simulink library "xbsIndex_r3"  (Simulink 6.1)
PreLoadFcn:
  | xlmeta;
undefined symbols (not defined in the file or in its folder): sim_pause
libraries: xbsIndex_r3 x62, simulink x1
(part 1 of 4)
settings Model: Creator=arvinds  LastModifiedBy=milne

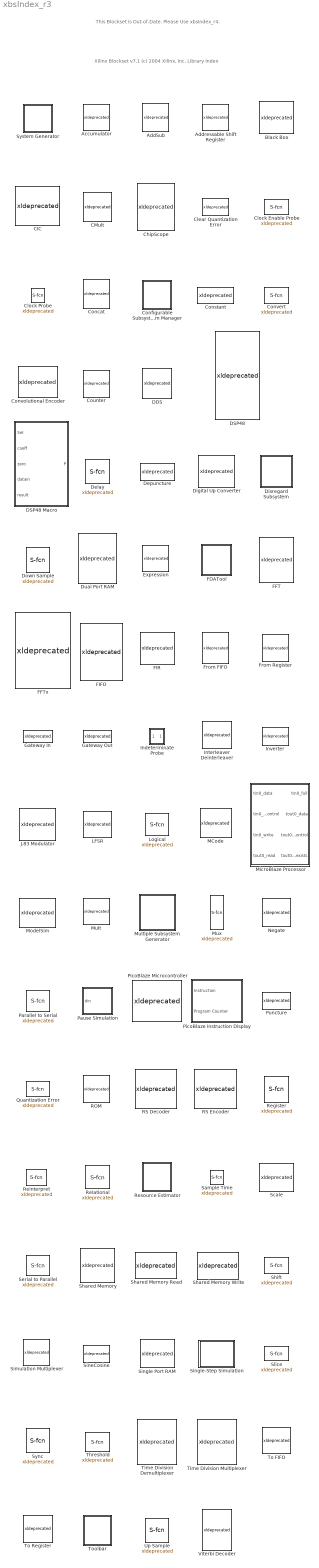
== system xbsIndex_r3 ==
  note: Xilinx Blockset v7.1
      | (c) 2004 Xilinx, Inc.
      |
      | Library Index
  note: This Blockset is Out-of-Date.
      | Please Use xbsIndex_r4.
  " System Generator" : Subsystem  Tag=genX  mask(Xilinx System Generator){xilinxfamily=Virtex2, part=xc2v1000, speed=-4, package=bg575, synthesis_tool=XST, directory=./netlist, testbench=off, simulink_period=1, sysclk_period=100, incr_netlist=off, trim_vbits=Everywhere in SubSystem, dbl_ovrd=According to Block Masks, core_generation=According to Block Masks, run_coregen=off, deprecated_control=off, eval_field=0}
      mask prompts: xilinxfamily "Xilinx Family"; synthesis_tool "Synthesis Tool"; directory "Target Directory"; simulink_period "Simulink Period"; sysclk_period "System Clock Period"; incr_netlist "Incremental Netlisting"; trim_vbits "Trim Valid Bits"; dbl_ovrd "Override with Doubles"; core_generation "Generate Cores"; run_coregen "Run CoreGen"; deprecated_control "Show Deprecated Controls"; eval_field "Evaluation Field"
      mask help: Interface to the Xilinx System Generator to generate HDL code for the subsystem hierarchy in which the block resides. The block also gives coarse grain (subsystem wide) control over capabilities such as overriding with doubles. Double click on the icon to access these features.
      mask init:
      | [bg,fg]=xlcmap_r3('SGen');
      | iPos = get_param(gcb,'Position');
      | iWidth=iPos(3)-iPos(1); iHeight=iPos(4)-iPos(2);
      | iCx=iWidth/2;
      | iCy=iHeight/2;
      | [logoX, logoY] = xlogo(iPos);
      settings: AttributesFormatString=System\nGenerator  OpenFcn=modelName = get_param(bdroot, 'name');h = errordlg(sprintf(['This block is from an outdated copy of the Xilinx Blockset.\nPlease run xlUpdateModel(''' modelName ''') to update this design.']), 'Update Required');
      mask Help: eval('xlWeb(xlhtmldoclink('' System Generator''))');
      mask StyleString: edit,edit,edit,edit,popup(Spectrum|Synplify|Synplify Pro|XST),edit,checkbox,edit,edit,checkbox,popup(According to Block Masks|Everywhere in SubSystem|No Where in SubSystem),popup(According to Block Masks|Everywhere in SubSystem|No Where in SubSystem),popup(According to Block Masks|Everywhere Available|Not Needed - Already Generated),checkbox,checkbox,edit
      mask Display:
      | patch([0 iWidth iWidth 0],[0 0 iHeight iHeight] , bg);
      | patch(logoX,logoY, fg);
      | ;plot([0 0 iWidth iWidth 0], [0 iHeight iHeight 0 0]);
  Accumulator : S-Function  FunctionName=xldeprecated  Parameters=nin,nout  mask(Xilinx Accumulator){n_bits=8, overflow=Wrap, operation=Add, scale=1, explicit_period=off, period=1, rst=on, hasbypass=off, en=off, dbl_ovrd=off, show_param=off, gen_core=off, use_rpm=on, xl_area=[0, 0, 0, 0, 0, 0, 0], xl_use_area=off}
      mask prompts: n_bits "Number of Output Bits"; scale "Feedback Scaling"; explicit_period "Use Explicit Sample Period"; period "Sample Period  (use -1 to inherit first known input period)"; rst "Provide Reset Port"; hasbypass "Reinitialize with Input 'b' on Reset"; en "Provide Enable Port"; dbl_ovrd "Override with Doubles"; show_param "---------------------- Show Implementation Parameters -----------------------------------------------------------------------------------"; gen_core "Generate Core"; use_rpm "Use Placement Information for Core"; xl_area "FPGA Area [Slices, FFs, BRAMs, LUTs, IOBs, Emb. Mults, TBUFs]"; xl_use_area "Use Area Above For Estimation"
      mask help:
      | BLOCK IS OUT OF DATE.
      |
      | This block is from an outdated copy of the Xilinx Blockset. Please run xlUpdateModel('<model-name>') to update to the latest version.
      mask init:
      | [designRoot, family, part, speed, package, simulinkPeriod, sysclkPeriod, dbl_ovrd, trimVbit] = xlSysgenSettings(gcb,1,1);
      | [bg,fg] = xlcmap_r3('XBlock',dbl_ovrd);
      | iPos = get_param(gcb,'Position');
      | iWidth=iPos(3)-iPos(1); iHeight=iPos(4)-iPos(2);
      | iCx=iWidth/2;
      | iCy=iHeight/2;
      | [logoX, logoY] = xlogo(iPos);
      | [enPortNum,enPortStr,rstPortNum,rstPortStr] = xlport_en_rst(en,rst,2);
      | 
      | % one time added for param list
      | hasRST = rst;
      | hasEN =  en;
      | dblOvrd = dbl_ovrd;
      | nbits = n_bits;
      | precision0 = 1;
      | useCore = 1;
      | gen_core = 1;
      | latency = 1;
      | explicitClk = explicit_period;
      | 
      | % just pass everything to s-function
      | sfcn_mwsv__ = get_param(gcb, 'MaskWSVariables');
      | 
      | nport = get_param(gcbh, 'ports');
      | nin = nport(1);
      | nout = nport(2);
      mask Help: eval('xlWeb(xlhtmldoclink(''Accumulator''))');
      mask StyleString: edit,popup(Wrap|Saturate|Error),popup(Add|Subtract),popup(1|1/2|1/4|1/8|1/16|1/32|1/64|1/128|1/256),checkbox,edit,checkbox,checkbox,checkbox,checkbox,checkbox,checkbox,checkbox,edit,checkbox
      mask Display:
      | patch([0 iWidth iWidth 0],[0 0 iHeight iHeight] , bg);
      | patch(logoX,logoY , fg);
      | port_label('output',1,'q');
      | port_label('input',1,'b');
      | port_label('input',enPortNum,enPortStr);
      | port_label('input',rstPortNum,rstPortStr);
      | ;plot([0 0 iWidth iWidth 0], [0 iHeight iHeight 0 0]);
  AddSub : S-Function  FunctionName=xldeprecated  Parameters=nin,nout  mask(Xilinx Adder/Subtractor){mode=Addition, precision=Full, arith_type=Unsigned, n_bits=8, bin_pt=2, quantization=Truncate, overflow=Wrap, latency=0, explicit_period=off, period=1, use_carryin=off, use_carryout=off, en=off, dbl_ovrd=off, show_param=off, use_core=on, pipeline=off, use_rpm=on, gen_core=off, xl_area=[0, 0, 0, 0, 0, 0, 0], xl_use_area=off}
      mask prompts: arith_type "Output Type"; n_bits "Number of Bits"; bin_pt "Binary Point"; explicit_period "Use Explicit Sample Period"; period "Sample Period  (use -1 to inherit first known input period)"; use_carryin "Provide Carry-in Port"; use_carryout "Provide Carry-out Port"; en "Provide Enable Port"; dbl_ovrd "Override with Doubles"; show_param "---------------------- Show Implementation Parameters -----------------------------------------------------------------------------------"; use_core "Implement with Xilinx Smart-IP Core"; pipeline "Pipeline to Greatest Extent Possible"; use_rpm "Use Placement Information for Core"; gen_core "Generate Core"; xl_area "FPGA Area [Slices, FFs, BRAMs, LUTs, IOBs, Emb. Mults, TBUFs]"; xl_use_area "Use Area Above For Estimation"
      mask help:
      | BLOCK IS OUT OF DATE.
      |
      | This block is from an outdated copy of the Xilinx Blockset. Please run xlUpdateModel('<model-name>') to update to the latest version.
      mask init:
      | rst = 0;
      | cin_port = 1; cin_str = 'a';
      | cout_port = 1; cout_str = '';
      | nextport = 3;
      | if(use_carryin)
      | 	cin_port = 3;
      | 	cin_str = 'cin';
      | 	nextport = 4;
      | end
      | if(use_carryout)
      | 	cout_port = 2;
      | 	cout_str = 'cout';
      | end
      | if (mode ~= 3)
      |    [enPortNum,enPortStr,rstPortNum,rstPortStr] = xlport_en_rst(en,rst,nextport);
      | else
      |   [enPortNum,enPortStr,rstPortNum,rstPortStr] = xlport_en_rst(en,rst,nextport+1);
      | end
      | 
      | [designRoot, family, part, speed, package, simulinkPeriod, sysclkPeriod, dbl_ovrd, trimVbit] = xlSysgenSettings(gcb,1,1);
      | mprt=1; mstr=''; ostr2='';
      | if (mode==1)
      |   ostr = 'a+b';
      | elseif (mode==2)
      |   ostr = 'a-b';
      | else
      |   ostr = 'a+b';
      |   ostr2 = '_b';
      |   if(use_carryin)
      |      mprt=4; 
      |   else
      | 	 mprt = 3;
      |   end
      |   mstr='sub';
      | end
      | zstr=''; zpstr='';
      | if latency > 0
      |   zstr = 'z';
      |   zpstr = sprintf('-%d', latency);
      | end
      | [bg,fg] = xlcmap_r3('XBlock',dbl_ovrd);
      | iPos = get_param(gcb,'Position');
      | iWidth=iPos(3)-iPos(1); iHeight=iPos(4)-iPos(2);
      | iCx=iWidth/2;
      | iCy=iHeight/2;
      | [logoX, logoY] = xlogo(iPos);
      | zstrx = 0.45*iWidth-3; if (zstrx<3) zstrx=3; end
      | zstry = 0.36*iHeight-7; if (zstry<3) zstry=3; end
      | 
      | 
      | % one time added for param list
      | dblOvrd = dbl_ovrd;
      | useCore = use_core;
      | precision0 = precision;
      | precision1 = precision;
      | z0 = [n_bits bin_pt arith_type quantization overflow];
      | z1 = [1 0 1 1 1];
      | explicitClk = explicit_period;
      | gen_core = 1;
      | hasRST = rst;
      | hasEN = en;
      | 
      | % just pass everything to s-function
      | sfcn_mwsv__ = get_param(gcb, 'MaskWSVariables');
      | 
      | nport = get_param(gcbh, 'ports');
      | nin = nport(1);
      | nout = nport(2);
      mask Help: eval('xlWeb(xlhtmldoclink(''AddSub''))');
      mask StyleString: popup(Addition|Subtraction|Addition or Subtraction),popup(Full|User Defined),popup(Unsigned|Signed  (2's comp)),edit,edit,popup(Truncate|Round  (unbiased: +/- Inf)),popup(Wrap|Saturate|Error),edit,checkbox,edit,checkbox,checkbox,checkbox,checkbox,checkbox,checkbox,checkbox,checkbox,checkbox,edit,checkbox
      mask Display:
      | patch([0 iWidth iWidth 0],[0 0 iHeight iHeight] , bg);
      | patch(logoX,logoY , fg);
      | text(zstrx,zstry,zstr);
      | text(zstrx+5,zstry+5,zpstr);
      | port_label('output',1,ostr);
      | port_label('output',1,ostr2);
      | port_label('output',cout_port,cout_str);
      | port_label('input',mprt,mstr)
      | port_label('input',1,'a');
      | port_label('input',2,'b');
      | port_label('input',cin_port,cin_str);
      | port_label('input',enPortNum,enPortStr);
      | ;plot([0 0 iWidth iWidth 0], [0 iHeight iHeight 0 0]);
  Addressable Shift Register : S-Function  FunctionName=xldeprecated  Parameters=nin,nout  mask(Xilinx Addressable Shift Register){infer_latency=on, depth=2, initVector=[0], explicit_period=off, period=1, accept_only_valid=off, en=off, dbl_ovrd=off, show_param=off, use_rpm=on, gen_core=off, xl_area=[0, 0, 0, 0, 0, 0, 0], xl_use_area=off}
      mask prompts: infer_latency "Infer Maximum Latency (depth) Using Address Port Width"; depth "Maximum Latency (depth)"; initVector "Initial Value Vector"; explicit_period "Use Explicit Sample Period"; period "Sample Period  (use -1 to inherit first known input period)"; accept_only_valid "Shift In Only Valid Data"; en "Provide Enable Port"; dbl_ovrd "Override with Doubles"; show_param "---------------------- Show Implementation Parameters -----------------------------------------------------------------------------------"; use_rpm "Use Placement Information for Core"; gen_core "Generate Core"; xl_area "FPGA Area [Slices, FFs, BRAMs, LUTs, IOBs, Emb. Mults, TBUFs]"; xl_use_area "Use Area Above For Estimation"
      mask help:
      | BLOCK IS OUT OF DATE.
      |
      | This block is from an outdated copy of the Xilinx Blockset. Please run xlUpdateModel('<model-name>') to update to the latest version.
      mask init:
      | % get enable port number and string
      | [enPortNum, enPortStr] =xlport_en_rst(en,0,3);
      | 
      | [designRoot, family, part, speed, package, simulinkPeriod, sysclkPeriod, dbl_ovrd, trimVbit] = xlSysgenSettings(gcb,1,1);
      | [bg,fg] = xlcmap_r3('XBlock',dbl_ovrd);
      | iPos = get_param(gcb,'Position');
      | iWidth=iPos(3)-iPos(1); iHeight=iPos(4)-iPos(2);
      | iCx=iWidth/2;
      | iCy=iHeight/2;
      | [logoX, logoY] = xlogo(iPos);
      | 
      | 
      | 
      | 
      | % one time added for param list
      | init = initVector;
      | useCore = 1;
      | dblOvrd = dbl_ovrd;
      | vOnly = accept_only_valid;
      | precision0 = 1;
      | explicitClk = explicit_period;
      | hasEN = en;
      | gen_core = 1;
      | rpm = use_rpm;
      | 
      | % just pass everything to s-function
      | sfcn_mwsv__ = get_param(gcb, 'MaskWSVariables');
      | 
      | nport = get_param(gcbh, 'ports');
      | nin = nport(1);
      | nout = nport(2);
      mask Help: eval('xlWeb(xlhtmldoclink(''Addressable Shift Register''))');
      mask Display:
      | patch([0 iWidth iWidth 0],[0 0 iHeight iHeight] , bg);
      | patch(logoX,logoY , fg);
      | port_label('input', 1,'d');
      | port_label('input', 2,'addr');
      | port_label('input',enPortNum,enPortStr);
      | port_label('output',1,'q');
      | 
      | ;plot([0 0 iWidth iWidth 0], [0 iHeight iHeight 0 0]);
  Black Box : S-Function  FunctionName=xldeprecated  Parameters=nin,nout  mask(Xilinx Blackbox Block){init_code=, sim_method=Inactive, engine_block=, show_param=off, xl_area=[0, 0, 0, 0, 0, 0, 0], xl_use_area=off}
      mask prompts: init_code "Block Configuration M-Function"; sim_method "Simulation Mode"; engine_block "HDL Co-Simulator To Use  (specify helper block by name)"; show_param "---------------------- Show Implementation Parameters -----------------------------------------------------------------------------------"; xl_area "FPGA Area [Slices, FFs, BRAMs, LUTs, IOBs, Emb. Mults, TBUFs]"; xl_use_area "Use Area Above For Estimation"
      mask help:
      | BLOCK IS OUT OF DATE.
      |
      | This block is from an outdated copy of the Xilinx Blockset. Please run xlUpdateModel('<model-name>') to update to the latest version.
      mask init:
      | [designRoot, family, part, speed, package, simulinkPeriod, sysclkPeriod, dbl_ovrd, trimVbit] = xlSysgenSettings(gcb,0,0);
      | 
      | [bg,fg] = xlcmap_r3('XBlock');
      | iPos = get_param(gcb,'Position');
      | iWidth=iPos(3)-iPos(1); iHeight=iPos(4)-iPos(2);
      | iCx=iWidth/2;
      | iCy=iHeight/2;
      | [logoX, logoY] = xlogo(iPos);
      | zstr='z'; zpstr='-1';
      | zstrx = iCx-3; if (zstrx<16) zstr='';zpstr=''; end
      | zstry = iCy;
      | 
      | precision0 = 1;
      | latency = 0;
      | dblOvrd = 0;
      | 
      | mdlPath = xlGetMdlDir(bdroot);
      | 
      | refBlk = get_param(gcb,'referenceBlock');
      | if (isempty(refBlk) | strncmp(refBlk,'xbsIndex',8))
      | 	srcPath = mdlPath;
      | else
      | 	srcPath = xlPathToReference;
      | 	if (isempty(srcPath))
      | 		srcPath = mdlPath;
      | 	end
      | end
      | 
      | if (sim_method==2)
      | 	validEngineBlock = 0;
      | 	try
      | 	  engineBlock = xlBlockNameRelPath(get_param(gcb,'Parent'),engine_block);
      | 	catch
      | 	  engineBlock = '//';
      | 	end
      | 	try 
      | 	  engineWorkDir = get_param(engineBlock,'dir');
      | 	  validEngineBlock = 1;
      | 	catch
      | 	end
      | end
      | 
      | % just pass everything to s-function
      | sfcn_mwsv__ = get_param(gcb, 'MaskWSVariables');
      | 
      | plabel = xlbbPortLabelStruct(gcb,init_code,mdlPath);
      | 
      | nport = get_param(gcbh, 'ports');
      | nin = nport(1);
      | nout = nport(2);
      mask Help: eval('xlWeb(xlhtmldoclink(''Black Box''))');
      mask StyleString: edit,popup(Inactive|Use HDL Co-Simulation),edit,checkbox,edit,checkbox
      mask Display:
      | patch([0 iWidth iWidth 0],[0 0 iHeight iHeight] , bg);
      | patch(logoX,logoY, fg);
      | plot([0 0 iWidth iWidth 0], [0 iHeight iHeight 0 0]);
      |   port_label(plabel.d1,plabel.i1,plabel.n1);
      |   port_label(plabel.d2,plabel.i2,plabel.n2);
      |   port_label(plabel.d3,plabel.i3,plabel.n3);
      |   port_label(plabel.d4,plabel.i4,plabel.n4);
      |   port_label(plabel.d5,plabel.i5,plabel.n5);
      |   port_label(plabel.d6,plabel.i6,plabel.n6);
      |   port_label(plabel.d7,plabel.i7,plabel.n7);
      |   port_label(plabel.d8,plabel.i8,plabel.n8);
      |   port_label(plabel.d9,plabel.i9,plabel.n9);
      |   port_label(plabel.d10,plabel.i10,plabel.n10);
      |   port_label(plabel.d11,plabel.i11,plabel.n11);
      |   port_label(plabel.d12,plabel.i12,plabel.n12);
      |   port_label(plabel.d13,plabel.i13,plabel.n13);
      |   port_label(plabel.d14,plabel.i14,plabel.n14);
      |   port_label(plabel.d15,plabel.i15,plabel.n15);
      |   port_label(plabel.d16,plabel.i16,plabel.n16);
      |   port_label(plabel.d17,plabel.i17,plabel.n17);
      |   port_label(plabel.d18,plabel.i18,plabel.n18);
      |   port_label(plabel.d19,plabel.i19,plabel.n19);
      |   port_label(plabel.d20,plabel.i20,plabel.n20);
      |   port_label(plabel.d21,plabel.i21,plabel.n21);
      |   port_label(plabel.d22,plabel.i22,plabel.n22);
      |   port_label(plabel.d23,plabel.i23,plabel.n23);
      |   port_label(plabel.d24,plabel.i24,plabel.n24);
      |   port_label(plabel.d25,plabel.i25,plabel.n25);
      |   port_label(plabel.d26,plabel.i26,plabel.n26);
      |   port_label(plabel.d27,plabel.i27,plabel.n27);
      |   port_label(plabel.d28,plabel.i28,plabel.n28);
      |   port_label(plabel.d29,plabel.i29,plabel.n29);
      |   port_label(plabel.d30,plabel.i30,plabel.n30);
      |   port_label(plabel.d31,plabel.i31,plabel.n31);
      |   port_label(plabel.d32,plabel.i32,plabel.n32);
      |   port_label(plabel.d33,plabel.i33,plabel.n33);
      |   port_label(plabel.d34,plabel.i34,plabel.n34);
      |   port_label(plabel.d35,plabel.i35,plabel.n35);
      |   port_label(plabel.d36,plabel.i36,plabel.n36);
      |   port_label(plabel.d37,plabel.i37,plabel.n37);
      |   port_label(plabel.d38,plabel.i38,plabel.n38);
      |   port_label(plabel.d39,plabel.i39,plabel.n39);
      |   port_label(plabel.d40,plabel.i40,plabel.n40);
      |   port_label(plabel.d41,plabel.i41,plabel.n41);
      |   port_label(plabel.d42,plabel.i42,plabel.n42);
      |   port_label(plabel.d43,plabel.i43,plabel.n43);
      |   port_label(plabel.d44,plabel.i44,plabel.n44);
      |   port_label(plabel.d45,plabel.i45,plabel.n45);
      |   port_label(plabel.d46,plabel.i46,plabel.n46);
      |   port_label(plabel.d45,plabel.i45,plabel.n45);
      |   port_label(plabel.d48,plabel.i48,plabel.n48);
      |   port_label(plabel.d49,plabel.i49,plabel.n49);
      |   port_label(plabel.d50,plabel.i50,plabel.n50);
      |   port_label(plabel.d51,plabel.i51,plabel.n51);
      |   port_label(plabel.d52,plabel.i52,plabel.n52);
      |   port_label(plabel.d53,plabel.i53,plabel.n53);
      |   port_label(plabel.d54,plabel.i54,plabel.n54);
      |   port_label(plabel.d55,plabel.i55,plabel.n55);
      |   port_label(plabel.d56,plabel.i56,plabel.n56);
      |   port_label(plabel.d57,plabel.i57,plabel.n57);
      |   port_label(plabel.d58,plabel.i58,plabel.n58);
      |   port_label(plabel.d59,plabel.i59,plabel.n59);
      |   port_label(plabel.d60,plabel.i60,plabel.n60);
      |   port_label(plabel.d61,plabel.i61,plabel.n61);
      |   port_label(plabel.d62,plabel.i62,plabel.n62);
      |   port_label(plabel.d63,plabel.i63,plabel.n63);
      |   port_label(plabel.d64,plabel.i64,plabel.n64);
  CIC : S-Function  FunctionName=xldeprecated  Parameters=nin,nout  mask(Xilinx Cascaded Integrator-Comb Filter){filter_type=Decimator, samp_rate_change=8, stages=2, differential_delay=1, latency=1, explicit_period=off, period=1, dbl_ovrd=off, show_param=off, use_rpm=on, gen_core=off, xl_area=[0, 0, 0, 0, 0, 0, 0], xl_use_area=off}
      mask prompts: filter_type "Filter Type"; samp_rate_change "Sample Rate Change"; stages "Number of Stages"; differential_delay "Differential Delay"; explicit_period "Use Explicit Sample Period"; period "Sample Period"; dbl_ovrd "Override with Doubles"; show_param "---------------------- Show Implementation Parameters -----------------------------------------------------------------------------------"; use_rpm "Use Placement Information for Core"; gen_core "Generate Core"; xl_area "FPGA Area [Slices, FFs, BRAMs, LUTs, IOBs, Emb. Mults, TBUFs]"; xl_use_area "Use Area Above For Estimation"
      mask help:
      | BLOCK IS OUT OF DATE.
      |
      | This block is from an outdated copy of the Xilinx Blockset. Please run xlUpdateModel('<model-name>') to update to the latest version.
      mask init:
      | [designRoot, family, part, speed, package, simulinkPeriod, sysclkPeriod, dbl_ovrd, trimVbit] = xlSysgenSettings(gcb,1,0);
      | trimVbit=1;
      | [bg,fg] = xlcmap_r3('XBlock',dbl_ovrd);
      | iPos = get_param(gcb,'Position');
      | iWidth=iPos(3)-iPos(1); iHeight=iPos(4)-iPos(2);
      | iCx=iWidth/2;
      | iCy=iHeight/2;
      | [logoX, logoY] = xlogo(iPos);
      | if(filter_type == 1)
      | str = sprintf('%d-Stage CIC\n1:%d Interpolator',stages,samp_rate_change);
      |      aw = 3;
      |      ah = 7;
      |      arrowX = [0, (-aw), (-aw), 0, 0, (1), (1), (aw+1), (aw+1), (1)];
      |      arrowY = [(ah-1), (ah-aw-1), (ah-aw), (ah), (-ah), (-ah), (ah), (ah-aw), (ah-aw-1),(ah-1)];
      |      arrowX = arrowX + iCx - 1 - 3.5*length(str);
      |      arrowY = arrowY + iCy + 3;
      | else
      | str = sprintf('%d-Stage CIC\n%d:1 Decimator',stages,samp_rate_change);
      |      aw = 3;
      |      ah = 7;
      |      arrowX = [0, (-aw), (-aw), 0, 0, (1), (1), (aw+1), (aw+1), (1)];
      |     arrowY = [(ah-1), (ah-aw-1), (ah-aw), (ah), (-ah), (-ah), (ah), (ah-aw), (ah-aw-1), (ah-1)];
      |     arrowX = arrowX + iCx - 2 - 3.5*length(str);
      |     arrowY = iCy - arrowY + 2;
      | end
      | 
      | % one time added for param list
      | rate_change = samp_rate_change;
      | diff_delay = differential_delay;
      | create_rpm = use_rpm;
      | dblOvrd = dbl_ovrd;
      | useCore = 1;
      | precision0 = 1;
      | precision1 = 1;
      | explicitClk = explicit_period;
      | gen_core = 1;
      | 
      | % just pass everything to s-function
      | sfcn_mwsv__ = get_param(gcb, 'MaskWSVariables');
      | 
      | nport = get_param(gcbh, 'ports');
      | nin = nport(1);
      | nout = nport(2);
      mask Help: eval('xlWeb(xlhtmldoclink(''CIC''))');
      mask StyleString: popup(Interpolator|Decimator),edit,edit,popup(1|2),edit,checkbox,edit,checkbox,checkbox,checkbox,checkbox,edit,checkbox
      mask Display:
      | patch([0 iWidth iWidth 0],[0 0 iHeight iHeight] , bg);
      | patch(logoX,logoY , fg);
      | disp(str);
      | plot([0 0 iWidth iWidth 0], [0 iHeight iHeight 0 0]);
      | 
      | port_label('input',1,'xn');
      | port_label('input',2,'vin');
      | 
      | port_label('output',1,'yn');
      | port_label('output',2,'vout');
  CMult : S-Function  FunctionName=xldeprecated  Parameters=nin,nout  mask(Xilinx Constant Multiplier){const=1, show_cparam=off, const_n_bits=8, const_bin_pt=6, show_output_param=off, precision=Full, arith_type=Signed  (2's comp), n_bits=8, bin_pt=6, quantization=Round  (unbiased: +/- Inf), overflow=Wrap, latency=0, explicit_period=off, period=1, en=off, dbl_ovrd=off, show_param=off, mult_type=Parallel, oversample=2, mem_type=Distributed RAM, pipeline=off, use_rpm=on, placement_style=Rectangular Shape, gen_core=off, xl_area=[0, 0, 0, 0, 0, 0, 0], xl_use_area=off}
      mask prompts: const "Value of Constant"; show_cparam "---------------------- Show Constant Data Type Parameters ---------------------------------------------------------"; const_n_bits "Number of Bits in Constant"; const_bin_pt "Binary Point of Constant"; show_output_param "---------------------- Show Output Data Type Parameters ------------------------------"; arith_type "Output Type"; n_bits "Number of Bits"; bin_pt "Binary Point"; explicit_period "Use Explicit Sample Period"; period "Sample Period  (use -1 to inherit first known input period)"; en "Provide Enable Port"; dbl_ovrd "Override with Doubles"; show_param "---------------------- Show Implementation Parameters -----------------------------------------------------------------------------------"; mult_type "Multiplier Type"; oversample "Hardware Over-Sampling Rate"; mem_type "Memory Type"; pipeline "Pipeline to Greatest Extent Possible"; use_rpm "Use Placement Information for Core"; placement_style "Placement Style"; gen_core "Generate Core"; xl_area "FPGA Area [Slices, FFs, BRAMs, LUTs, IOBs, Emb. Mults, TBUFs]"; xl_use_area "Use Area Above For Estimation"
      mask help:
      | BLOCK IS OUT OF DATE.
      |
      | This block is from an outdated copy of the Xilinx Blockset. Please run xlUpdateModel('<model-name>') to update to the latest version.
      mask init:
      | rst = 0;
      | [enPortNum,enPortStr,rstPortNum,rstPortStr] = xlport_en_rst(en,rst,2);
      | 
      | multtype = mult_type;
      | if (multtype == 2)
      |   osamp = oversample;
      | else
      |   osamp = 1;
      | end
      | mprt = 1; ostr='';
      | mprt_loadb = 1; ostr_loadb='';
      | const_arith_type = (const<0) + 1;
      | [designRoot, family, part, speed, package, simulinkPeriod, sysclkPeriod, dbl_ovrd, trimVbit] = xlSysgenSettings(gcb,1,1);
      | k = xltodouble(const, const_n_bits, const_bin_pt, const_arith_type, 2, 2);
      | if (k<0)
      |   str = sprintf('x (%0.4g)',k);
      | else
      |   str = sprintf('x %0.4g',k);
      | end
      | zstr=''; zpstr='';
      | if latency > 0
      |   zstr = 'z';
      |   zpstr = sprintf('-%d', latency);
      | end
      | [bg,fg] = xlcmap_r3('XBlock',dbl_ovrd);
      | iPos = get_param(gcb,'Position');
      | iWidth=iPos(3)-iPos(1); iHeight=iPos(4)-iPos(2);
      | iCx=iWidth/2;
      | iCy=iHeight/2;
      | [logoX, logoY] = xlogo(iPos);
      | logoX = logoX*.54 + 2;
      | logoY = logoY*.54+ iHeight*.23;
      | zstrx = 15;
      | zstry = 0.36*iHeight-4; if (zstry<3) zstry=3; end
      | 
      | 
      | 
      | % one time added for param list
      | dblOvrd = dbl_ovrd;
      | useCore = 1;
      | precision0 = precision;
      | z0 = [n_bits bin_pt arith_type quantization overflow];
      | coef = const;
      | ctype = [const_n_bits const_bin_pt const_arith_type 2 2];
      | explicitClk = explicit_period;
      | memtype = mem_type;
      | reload = 0;
      | oversample = osamp;
      | gen_core = 1;
      | rpm = use_rpm;
      | style = placement_style;
      | hasRST = rst;
      | hasEN = en;
      | 
      | % just pass everything to s-function
      | sfcn_mwsv__ = get_param(gcb, 'MaskWSVariables');
      | 
      | nport = get_param(gcbh, 'ports');
      | nin = nport(1);
      | nout = nport(2);
      mask Help: eval('xlWeb(xlhtmldoclink(''CMult''))');
      mask StyleString: edit,checkbox,edit,edit,checkbox,popup(Full|User Defined),popup(Unsigned|Signed  (2's comp)),edit,edit,popup(Truncate|Round  (unbiased: +/- Inf)),popup(Wrap|Saturate|Flag as Error),edit,checkbox,edit,checkbox,checkbox,checkbox,popup(Parallel|Sequential),edit,popup(Distributed RAM|Block RAM),checkbox,checkbox,popup(Rectangular Shape|Triangular Packing),checkbox,edit,checkbox
      mask Display:
      | patch([0 iWidth 0],[0 iCy iHeight] , bg);
      | patch(logoX,logoY , fg);
      | plot([0 iWidth 0 0],[0 iCy iHeight 0] );
      | text(zstrx,zstry,zstr);
      | text(zstrx+4,zstry+4,zpstr);
      | port_label('output',1,[str  '  ']);
      | port_label('input',enPortNum,enPortStr);
  ChipScope : S-Function  Tag=chipScopeGenerate  FunctionName=xldeprecated  Parameters=nin,nout  mask(Xilinx ChipScope Core){num_trig_ports=2, show_trig_port=0, match_units_t0=1, match_type_t0=Basic, match_units_t1=1, match_type_t1=Basic, match_units_t2=1, match_type_t2=Basic, match_units_t3=1, match_type_t3=Basic, match_units_t4=1, match_type_t4=Basic, match_units_t5=1, match_type_t5=Basic, match_units_t6=1, match_type_t6=Basic, match_units_t7=1, match_type_t7=Basic, match_units_t8=1, match_type_t8=Basic, match_units_t9=3, match_type_t9=Basic, match_units_t10=1, match_type_t10=Basic, match_units_t11=1, match_type_t11=Basic, match_units_t12=1, match_type_t12=Basic, match_units_t13=1, match_type_t13=Basic, match_units_t14=1, match_type_t14=Basic, match_units_t15=1, match_type_t15=Basic, data_is_trigger=off, num_data_ports=1, data_depth=512, SRL16s=on, explicit_period=off, period=-1, dbl_ovrd=off}
      mask prompts: num_trig_ports "Number of Trigger Ports"; show_trig_port "Display Options for Trigger Port"; match_units_t0 "Number of Match Units for Trigger Port 0"; match_type_t0 "Match Type of Trigger Port 0"; match_units_t1 "Number of Match Units for Trigger Port 1"; match_type_t1 "Match Type of Trigger Port 1"; match_units_t2 "Number of Match Units for Trigger Port 2"; match_type_t2 "Match Type of Trigger Port 2"; match_units_t3 "Number of Match Units for Trigger Port 3"; match_type_t3 "Match Type of Trigger Port 3"; match_units_t4 "Number of Match Units for Trigger Port 4"; match_type_t4 "Match Type of Trigger Port 4"; match_units_t5 "Number of Match Units for Trigger Port 5"; match_type_t5 "Match Type of Trigger Port 5"; match_units_t6 "Number of Match Units for Trigger Port 6"; match_type_t6 "Match Type of Trigger Port 6"; match_units_t7 "Number of Match Units for Trigger Port 7"; match_type_t7 "Match Type of Trigger Port 7"; match_units_t8 "Number of Match Units for Trigger Port 8"; match_type_t8 "Match Type of Trigger Port 8"; match_units_t9 "Number of Match Units for Trigger Port 9"; match_type_t9 "Match Type of Trigger Port 9"; match_units_t10 "Number of Match Units for Trigger Port 10"; match_type_t10 "Match Type of Trigger Port 10"; match_units_t11 "Number of Match Units for Trigger Port 11"; match_type_t11 "Match Type of Trigger Port 11"; match_units_t12 "Number of Match Units for Trigger Port 12"; match_type_t12 "Match Type of Trigger Port 12"; match_units_t13 "Number of Match Units for Trigger Port 13"; match_type_t13 "Match Type of Trigger Port 13"; match_units_t14 "Number of Match Units for Trigger Port 14"; match_type_t14 "Match Type of Trigger Port 14"; match_units_t15 "Number of Match Units for Trigger Port 15"; match_type_t15 "Match Type of Trigger Port 15"; data_is_trigger "Use Trigger Ports as Data"; num_data_ports "Number of Data Ports"; data_depth "Depth of Capture Buffer"; SRL16s "Use SRL16s ( when possible)"; explicit_period "Use Explicit Sample Period"; period "Sample Period  (use -1 to inherit first known input period)"; dbl_ovrd "Override with Doubles"
      mask help:
      | BLOCK IS OUT OF DATE.
      |
      | This block is from an outdated copy of the Xilinx Blockset. Please run xlUpdateModel('<model-name>') to update to the latest version.
      mask init:
      | try
      | 
      | [designRoot, family, part, speed, package, simulinkPeriod, sysclkPeriod, dbl_ovrd, trimVbit] = xlSysgenSettings(gcb,1,1);
      | if isempty(family)
      | 	family = 'Virtex2';
      | end;
      | [xldirectory, xlSynthTool] = xlFindTargetDir(gcb);
      | xlISEVer = xlGetISEVer;
      | sysgen_root = fileparts(fileparts(which('sysgen')));
      | 
      | [bg,fg] = xlcmap_r3('XBlock',dbl_ovrd);
      | iPos = get_param(gcb,'Position');
      | iWidth=iPos(3)-iPos(1); iHeight=iPos(4)-iPos(2);
      | iCx=iWidth/2;
      | iCy=iHeight/2;
      | [logoX, logoY] = xlogo(iPos);
      | 
      | if (data_is_trigger == 1)
      | 	numDataPorts = 0;
      | else
      | 	numDataPorts = num_data_ports;
      | end;
      | inputs = num_trig_ports + numDataPorts;
      | dprt = [1:inputs ones(1,144-inputs)];
      | for i = 1:144
      | 	dstr{i} = ''; 
      | end;
      | 
      | % Set trigger port names
      | for i = 1:num_trig_ports
      | 	if (data_is_trigger == 1)
      | 		dstr{i} = ['trig' num2str(i-1) '/data' num2str(i-1)];
      | 	else
      | 		dstr{i} = ['trig' num2str(i-1)]; 
      | 	end;
      | end;
      | 
      | % Set data port names
      | for i = 1:numDataPorts
      | 	dstr{i+num_trig_ports} = ['data' num2str(i-1)];
      | end;
      | 
      | % Replace default names with signal names
      | signalNames = xlInputSignalNames(gcb);
      | for i = 1:length(signalNames)
      | 	if ~isempty(signalNames{i})
      | 		dstr{i} = signalNames{i};
      | 	end;
      | end;
      | 
      | % one time added for param list
      | latency = 1;
      | precision0 = 1;
      | dblOvrd = 0;
      | 
      | % just pass everything to s-function
      | sfcn_mwsv__ = get_param(gcb, 'MaskWSVariables');
      | 
      | catch
      | 	disp(lasterr);
      | end;
      | nport = get_param(gcbh, 'ports');
      | nin = nport(1);
      | nout = nport(2);
      mask Help: eval('xlWeb(xlhtmldoclink(''ChipScope''))');
      mask StyleString: popup(1|2|3|4|5|6|7|8|9|10|11|12|13|14|15|16),popup(0|1|2|3|4|5|6|7|8|9|10|11|12|13|14|15),popup(1|2|3|4),popup(Basic|Basic With Edges|Extended|Extended With Edges|Range|Range With Edges),popup(1|2|3|4),popup(Basic|Basic With Edges|Extended|Extended With Edges|Range|Range With Edges),popup(1|2|3|4),popup(Basic|Basic With Edges|Extended|Extended With edges|Range|Range With Edges),popup(1|2|3|4),popup(Basic|Basic With Edges|Extended|Extended With Edges|Range|Range With Edges),popup(1|2|3|4),popup(Basic|Basic With Edges|Extended|Extended With Edges|Range|Range With Edges),popup(1|2|3|4),popup(Basic|Basic With Edges|Extended|Extended With Edges|Range|Range with Edges),popup(1|2|3|4),popup(Basic|Basic With Edges|Extended|Extended With Edges|Range|Range With Edges),popup(1|2|3|4),popup(Basic|Basic With Edges|Extended|Extended With Edges|Range|Range With Edges),popup(1|2|3|4),popup(Basic|Basic With Edges|Extended|Extended With Edges|Range|Range With Edges),popup(1|2|3|4),popup(Basic|Basic With Edges|Extended|Extended With Edges|Range|Range With Edges),popup(1|2|3|4),popup(Basic|Basic With Edges|Extended|Extended with Edges|Range|Range With Edges),popup(1|2|3|4),popup(Basic|Basic With Edges|Extended|Extended With Edges|Range|Range With Edges),popup(1|2|3|4),popup(Basic|Basic With Edges|Extended|Extended With Edges|Range|Range With Edges),popup(1|2|3|4),popup(Basic|Basic With Edges|Extended|Extended With Edges|Range|Range With Edges),popup(1|2|3|4),popup(Basic|Basic With Edges|Extended|Extended With Edges|Range|Range With Edges),popup(1|2|3|4),popup(Basic|Basic With edges|Extended|Extended With Edges|Range|Range With Edges),checkbox,edit,popup(512|1024|2048|4096|8192|16384),checkbox,checkbox,edit,checkbox
      mask Display:
      | patch([0 iWidth iWidth 0],[0 0 iHeight iHeight] , bg);
      | patch(logoX,logoY, fg);
      | ;plot([0 0 iWidth iWidth 0], [0 iHeight iHeight 0 0]);
      | 
      | port_label('input',dprt(1),dstr{1});
      | port_label('input',dprt(2),dstr{2});
      | port_label('input',dprt(3),dstr{3});
      | port_label('input',dprt(4),dstr{4});
      | port_label('input',dprt(5),dstr{5});
      | port_label('input',dprt(6),dstr{6});
      | port_label('input',dprt(7),dstr{7});
      | port_label('input',dprt(8),dstr{8});
      | port_label('input',dprt(9),dstr{9});
      | port_label('input',dprt(10),dstr{10});
      | port_label('input',dprt(11),dstr{11});
      | port_label('input',dprt(12),dstr{12});
      | port_label('input',dprt(13),dstr{13});
      | port_label('input',dprt(14),dstr{14});
      | port_label('input',dprt(15),dstr{15});
      | port_label('input',dprt(16),dstr{16});
      | port_label('input',dprt(17),dstr{17});
      | port_label('input',dprt(18),dstr{18});
      | port_label('input',dprt(19),dstr{19});
      | port_label('input',dprt(20),dstr{20});
      | port_label('input',dprt(21),dstr{21});
      | port_label('input',dprt(22),dstr{22});
      | port_label('input',dprt(23),dstr{23});
      | port_label('input',dprt(24),dstr{24});
      | port_label('input',dprt(25),dstr{25});
      | port_label('input',dprt(26),dstr{26});
      | port_label('input',dprt(27),dstr{27});
      | port_label('input',dprt(28),dstr{28});
      | port_label('input',dprt(29),dstr{29});
      | port_label('input',dprt(30),dstr{30});
      | port_label('input',dprt(31),dstr{31});
      | port_label('input',dprt(32),dstr{32});
      | port_label('input',dprt(33),dstr{33});
      | port_label('input',dprt(34),dstr{34});
      | port_label('input',dprt(35),dstr{35});
      | port_label('input',dprt(36),dstr{36});
      | port_label('input',dprt(37),dstr{37});
      | port_label('input',dprt(38),dstr{38});
      | port_label('input',dprt(39),dstr{39});
      | port_label('input',dprt(40),dstr{40});
      | port_label('input',dprt(41),dstr{41});
      | port_label('input',dprt(42),dstr{42});
      | port_label('input',dprt(43),dstr{43});
      | port_label('input',dprt(44),dstr{44});
      | port_label('input',dprt(45),dstr{45});
      | port_label('input',dprt(46),dstr{46});
      | port_label('input',dprt(47),dstr{47});
      | port_label('input',dprt(48),dstr{48});
      | port_label('input',dprt(49),dstr{49});
      | port_label('input',dprt(50),dstr{50});
      | port_label('input',dprt(51),dstr{51});
      | port_label('input',dprt(52),dstr{52});
      | port_label('input',dprt(53),dstr{53});
      | port_label('input',dprt(54),dstr{54});
      | port_label('input',dprt(55),dstr{55});
      | port_label('input',dprt(56),dstr{56});
      | port_label('input',dprt(57),dstr{57});
      | port_label('input',dprt(58),dstr{58});
      | port_label('input',dprt(59),dstr{59});
      | port_label('input',dprt(60),dstr{60});
      | port_label('input',dprt(61),dstr{61});
      | port_label('input',dprt(62),dstr{62});
      | port_label('input',dprt(63),dstr{63});
      | port_label('input',dprt(64),dstr{64});
      | port_label('input',dprt(65),dstr{65});
      | port_label('input',dprt(66),dstr{66});
      | port_label('input',dprt(67),dstr{67});
      | port_label('input',dprt(68),dstr{68});
      | port_label('input',dprt(69),dstr{69});
      | port_label('input',dprt(70),dstr{70});
      | port_label('input',dprt(71),dstr{71});
      | port_label('input',dprt(72),dstr{72});
      | port_label('input',dprt(73),dstr{73});
      | port_label('input',dprt(74),dstr{74});
      | port_label('input',dprt(75),dstr{75});
      | port_label('input',dprt(76),dstr{76});
      | port_label('input',dprt(77),dstr{77});
      | port_label('input',dprt(78),dstr{78});
      | port_label('input',dprt(79),dstr{79});
      | port_label('input',dprt(80),dstr{80});
      | port_label('input',dprt(81),dstr{81});
      | port_label('input',dprt(82),dstr{82});
      | port_label('input',dprt(83),dstr{83});
      | port_label('input',dprt(84),dstr{84});
      | port_label('input',dprt(85),dstr{85});
      | port_label('input',dprt(86),dstr{86});
      | port_label('input',dprt(87),dstr{87});
      | port_label('input',dprt(88),dstr{88});
      | port_label('input',dprt(89),dstr{89});
      | port_label('input',dprt(90),dstr{90});
      | port_label('input',dprt(91),dstr{91});
      | port_label('input',dprt(92),dstr{92});
      | port_label('input',dprt(93),dstr{93});
      | port_label('input',dprt(94),dstr{94});
      | port_label('input',dprt(95),dstr{95});
      | port_label('input',dprt(96),dstr{96});
      | port_label('input',dprt(97),dstr{97});
      | port_label('input',dprt(98),dstr{98});
      | port_label('input',dprt(99),dstr{99});
      | port_label('input',dprt(100),dstr{100});
      | port_label('input',dprt(101),dstr{101});
      | port_label('input',dprt(102),dstr{102});
      | port_label('input',dprt(103),dstr{103});
      | port_label('input',dprt(104),dstr{104});
      | port_label('input',dprt(105),dstr{105});
      | port_label('input',dprt(106),dstr{106});
      | port_label('input',dprt(107),dstr{107});
      | port_label('input',dprt(108),dstr{108});
      | port_label('input',dprt(109),dstr{109});
      | port_label('input',dprt(110),dstr{110});
      | port_label('input',dprt(111),dstr{111});
      | port_label('input',dprt(112),dstr{112});
      | port_label('input',dprt(113),dstr{113});
      | port_label('input',dprt(114),dstr{114});
      | port_label('input',dprt(115),dstr{115});
      | port_label('input',dprt(116),dstr{116});
      | port_label('input',dprt(117),dstr{117});
      | port_label('input',dprt(118),dstr{118});
      | port_label('input',dprt(119),dstr{119});
      | port_label('input',dprt(120),dstr{120});
      | port_label('input',dprt(121),dstr{121});
      | port_label('input',dprt(122),dstr{122});
      | port_label('input',dprt(123),dstr{123});
      | port_label('input',dprt(124),dstr{124});
      | port_label('input',dprt(125),dstr{125});
      | port_label('input',dprt(126),dstr{126});
      | port_label('input',dprt(127),dstr{127});
      | port_label('input',dprt(128),dstr{128});
      | port_label('input',dprt(129),dstr{129});
      | port_label('input',dprt(130),dstr{130});
      | port_label('input',dprt(131),dstr{131});
      | port_label('input',dprt(132),dstr{132});
      | port_label('input',dprt(133),dstr{133});
      | port_label('input',dprt(134),dstr{134});
      | port_label('input',dprt(135),dstr{135});
      | port_label('input',dprt(136),dstr{136});
      | port_label('input',dprt(137),dstr{137});
      | port_label('input',dprt(138),dstr{138});
      | port_label('input',dprt(139),dstr{139});
      | port_label('input',dprt(140),dstr{140});
      | port_label('input',dprt(141),dstr{141});
      | port_label('input',dprt(142),dstr{142});
      | port_label('input',dprt(143),dstr{143});
      | port_label('input',dprt(144),dstr{144});
  Clear Quantization Error : S-Function  FunctionName=xldeprecated  Parameters=nin,nout  mask(Xilinx Clear Quantization Error Block){opt_port=off}
      mask prompts: opt_port "Add Optional Clear Port"
      mask help:
      | BLOCK IS OUT OF DATE.
      |
      | This block is from an outdated copy of the Xilinx Blockset. Please run xlUpdateModel('<model-name>') to update to the latest version.
      mask init:
      | [designRoot, family, part, speed, package, simulinkPeriod, sysclkPeriod, dbl_ovrd, trimVbit] = xlSysgenSettings(gcb,0,2);
      | [bg,fg] = xlcmap_r3('XBlock',dbl_ovrd);
      | iPos = get_param(gcb,'Position');
      | iWidth=iPos(3)-iPos(1); iHeight=iPos(4)-iPos(2);
      | iCx=iWidth/2;
      | iCy=iHeight/2;
      | [logoX, logoY] = xlogo(iPos);
      | if (opt_port==0)
      |   pnum=1;
      |   pstr='';
      | else
      |   pnum=2;
      |   pstr='*clrE';
      | end
      | 
      | % one time added for param list
      | precision0 = 1;
      | has_clr_pin = opt_port;
      | dblOvrd = dbl_ovrd;
      | 
      | % just pass everything to s-function
      | sfcn_mwsv__ = get_param(gcb, 'MaskWSVariables');
      | 
      | nport = get_param(gcbh, 'ports');
      | nin = nport(1);
      | nout = nport(2);
      mask Help: eval('xlWeb(xlhtmldoclink(''Clear Quantization Error''))');
      mask Display:
      | patch([0 iWidth iWidth 0],[0 0 iHeight iHeight] , bg);
      | patch(logoX,logoY , fg);
      | port_label('input',pnum,pstr);
      | port_label('output',1,'clr err');
      | ;plot([0 0 iWidth iWidth 0], [0 iHeight iHeight 0 0]);
  Clock Enable Probe : S-Function  FunctionName=xldeprecated  Parameters=nin,nout  mask(Xilinx Clock Enable Probe){}
      mask help:
      | BLOCK IS OUT OF DATE.
      |
      | This block is from an outdated copy of the Xilinx Blockset. Please run xlUpdateModel('<model-name>') to update to the latest version.
      mask init:
      | [designRoot, family, part, speed, package, simulinkPeriod, sysclkPeriod] = xlSysgenSettings(gcb,0,0);
      | 
      | [bg,fg] = xlcmap_r3('XBlock',0);
      | iPos = get_param(gcb,'Position');
      | iWidth=iPos(3)-iPos(1); iHeight=iPos(4)-iPos(2);
      | iCx=iWidth/2;
      | iCy=iHeight/2;
      | [logoX, logoY] = xlogo(iPos);
      | 
      | % one time added for param list
      | precision0 = 1;
      | dblOvrd = 0;
      | trimVbit = 0;
      | 
      | % just pass everything to s-function
      | sfcn_mwsv__ = get_param(gcb, 'MaskWSVariables');
      | 
      | nport = get_param(gcbh, 'ports');
      | nin = nport(1);
      | nout = nport(2);
      mask Help: eval('xlWeb(xlhtmldoclink(''Clock Enable Probe''))');
      mask Display:
      | patch([0 iWidth iWidth 0],[0 0 iHeight iHeight] , bg);
      | patch(logoX,logoY, fg);
      | ;plot([0 0 iWidth iWidth 0], [0 iHeight iHeight 0 0]);
      | 
      | disp('CE');
  Clock Probe : S-Function  FunctionName=xldeprecated  Parameters=nin,nout  mask(Xilinx Clock Probe){}
      mask help:
      | BLOCK IS OUT OF DATE.
      |
      | This block is from an outdated copy of the Xilinx Blockset. Please run xlUpdateModel('<model-name>') to update to the latest version.
      mask init:
      | [designRoot, family, part, speed, package, simulinkPeriod, sysclkPeriod, dbl_ovrd, trimVbit] = xlSysgenSettings(gcb,0,0);
      | 
      | [bg,fg] = xlcmap_r3('IO');
      | iPos = get_param(gcb,'Position');
      | iWidth=iPos(3)-iPos(1); iHeight=iPos(4)-iPos(2);
      | iCx=iWidth/2;
      | iCy=iHeight/2;
      | shapeX = iCx* (1 + cos(0:pi/6:2*pi));
      | shapeY = iCy* (1 + sin(0:pi/6:2*pi));
      | 
      | % just pass everything to s-function
      | sfcn_mwsv__ = get_param(gcb, 'MaskWSVariables');
      | 
      | nport = get_param(gcbh, 'ports');
      | nin = nport(1);
      | nout = nport(2);
      mask Help: eval('xlWeb(xlhtmldoclink(''Clock Probe''))');
      mask Display:
      | patch(shapeX,shapeY, bg);
      | plot(shapeX,shapeY);
      | disp('CLK');
  Concat : S-Function  FunctionName=xldeprecated  Parameters=nin,nout  mask(Xilinx Bus Concatenator){num_inputs=2, explicit_period=off, period=1, dbl_ovrd=off}
      mask prompts: num_inputs "Number of Inputs"; explicit_period "Use Explicit Sample Period"; period "Sample Period  (use -1 to inherit first known input period)"; dbl_ovrd "Override with Doubles"
      mask help:
      | BLOCK IS OUT OF DATE.
      |
      | This block is from an outdated copy of the Xilinx Blockset. Please run xlUpdateModel('<model-name>') to update to the latest version.
      mask init:
      | [designRoot, family, part, speed, package, simulinkPeriod, sysclkPeriod, dbl_ovrd, trimVbit] = xlSysgenSettings(gcb,1,1);
      | [bg,fg] = xlcmap_r3('XBlock',dbl_ovrd);
      | iPos = get_param(gcb,'Position');
      | iWidth=iPos(3)-iPos(1); iHeight=iPos(4)-iPos(2);
      | iCx=iWidth/2;
      | iCy=iHeight/2;
      | [logoX, logoY] = xlogo(iPos);
      | 
      | 
      | 
      | 
      | % one time added for param list
      | numInputs = num_inputs + 1;
      | precision0 = 1;
      | latency = 0;
      | dblOvrd = dbl_ovrd;
      | explicitClk = explicit_period;
      | 
      | 
      | % just pass everything to s-function
      | sfcn_mwsv__ = get_param(gcb, 'MaskWSVariables');
      | 
      | nport = get_param(gcbh, 'ports');
      | nin = nport(1);
      | nout = nport(2);
      mask Help: eval('xlWeb(xlhtmldoclink(''Concat''))');
      mask StyleString: popup(2|3|4|5|6|7|8|9|10|11|12|13|14|15|16),checkbox,edit,checkbox
      mask Display:
      | patch([0 iWidth iWidth 0],[0 0 iHeight iHeight] , bg);
      | patch(logoX,logoY, fg);
      | port_label('input',1,'hi');
      | port_label('input',num_inputs+1,'lo');
      | port_label('output',1,'cat');
      | ;plot([0 0 iWidth iWidth 0], [0 iHeight iHeight 0 0]);
  Configurable Subsystem Manager : Subsystem  Tag=xcfgMgr  mask(Xilinx System Generator){}
      mask help: Interface to the Xilinx System Generator to generate HDL code for the subsystem hierarchy in which the block resides. The block also gives coarse grain (subsystem wide) control over capabilities such as overriding with doubles. Double click on the icon to access these features.
      mask init:
      | [bg, fg] = xlcmap_r3('XTool');
      | 
      | %[bg1, fg] = xlcmap_r3('XBlock',0);
      | iPos = get_param(gcb,'Position');
      | iWidth=iPos(3)-iPos(1); iHeight=iPos(4)-iPos(2);
      | iCx=iWidth/2;
      | iCy=iHeight/2;
      | [logoX, logoY] = xlogo(iPos);
      settings: AttributesFormatString=Configurable Subsystem\nManager  OpenFcn=modelName = get_param(bdroot, 'name');h = errordlg(sprintf(['This block is from an outdated copy of the Xilinx Blockset.\nPlease run xlUpdateModel(''' modelName ''') to update this design.']), 'Update Required');
      mask Help: eval('xlWeb(xlhtmldoclink(''Configurable Subsystem Manager''))');
      mask Display:
      | patch([0 iWidth iWidth 0],[0 0 iHeight iHeight] , bg);
      | patch(logoX,logoY , fg);
      | ;plot([0 0 iWidth iWidth 0], [0 iHeight iHeight 0 0]);
  Constant : S-Function  FunctionName=xldeprecated  Parameters=nin,nout  mask(Xilinx Constant Block){const=1, equ=P=C, arith_type=Unsigned, n_bits=1, bin_pt=0, opselect=C, inp2=PCIN>>17, opr=+, inp1=P, carry=CIN, iostate=0, explicit_period=off, period=1, dbl_ovrd=off}
      mask prompts: const "Constant Value"; equ "DSP48 operation"; arith_type "Type"; n_bits "Number of Bits"; bin_pt "Binary Point Position"; opselect "Operation Select"; inp2 "Z Mux"; opr "Operand"; inp1 "YX Muxes"; carry "Carry Input"; explicit_period "Sampled Constant"; period "Sample Period"; dbl_ovrd "Override with Double"
      mask help:
      | BLOCK IS OUT OF DATE.
      |
      | This block is from an outdated copy of the Xilinx Blockset. Please run xlUpdateModel('<model-name>') to update to the latest version.
      mask init:
      | [designRoot, family, part, speed, package, simulinkPeriod, sysclkPeriod, dbl_ovrd, trimVbit] = xlSysgenSettings(gcb,1,2);
      | [bg,fg]=xlcmap_r3('XBlock',dbl_ovrd);
      | iPos = get_param(gcb,'Position');
      | iWidth=iPos(3)-iPos(1); iHeight=iPos(4)-iPos(2);
      | nchar = floor(iWidth/7.0);
      | op = 0;
      | dsp48instr = 0;
      | if (arith_type==1)
      |   bool = 1;
      |   k= xltodouble(const,1,0,1,2,2);
      |   format_str = sprintf('%%0.%dg',nchar);
      |   str = sprintf(format_str,k);
      |   if (length(str)+3<nchar)
      |   	str = ['k =' str];
      |   end
      | elseif (arith_type == 4) %dsp48
      |   dsp48instr = 1;
      |   bool = 0;
      |   str = equ;
      |   n_bits = 11;
      |   bin_pt = 0;
      |   arith_type = 1;
      |   [op,opmode, sub, carryin, carryin_sel] = xlcalcDSP48Op(equ);
      | else
      |   bool = 0;
      |   arith_type=arith_type-1;
      |   k= xltodouble(const,n_bits,bin_pt,arith_type,2,2);
      |   format_str = sprintf('%%0.%dg',nchar);
      |   str = sprintf(format_str,k);
      |   if (length(str)+3<nchar)
      |     str = ['k =' str];
      |   end
      | end
      | 
      | 
      | iCx=iWidth/2;
      | iCy=iHeight/2;
      | [logoX, logoY] = xlogo(iPos);
      | 
      | 
      | % one time added for param list
      | dblOvrd = dbl_ovrd;
      | precision0 = 2;
      | z0 = [n_bits bin_pt arith_type 2 2];
      | explicitClk = explicit_period;
      | 
      | 
      | % just pass everything to s-function
      | sfcn_mwsv__ = get_param(gcb, 'MaskWSVariables');
      | 
      | nport = get_param(gcbh, 'ports');
      | nin = nport(1);
      | nout = nport(2);
      mask Help: eval('xlWeb(xlhtmldoclink(''Constant''))');
      mask StyleString: edit,edit,popup(Boolean|Unsigned|Signed  (2's comp)|DSP48 Instruction),edit,edit,popup(C + A*B|PCIN + A*B|P + A*B|A * B|C + A:B|C - A:B|C|custom),popup(0|PCIN|P|C|PCIN>>17|P>>17),popup(+|-),popup(0|P|A:B|A*B|C|P+C|A:B+C),popup(0|1|CIN|~SIGN(P or PCIN)|~SIGN(A*B or A:B)|~SIGND(A*B or A:B)),edit,checkbox,edit,checkbox
      mask Display:
      | patch([0 iWidth iWidth 0],[0 0 iHeight iHeight] , bg);
      | patch(logoX,logoY , fg);
      | port_label('output',1,str);
      | ;plot([0 0 iWidth iWidth 0], [0 iHeight iHeight 0 0]);
  Convert : S-Function  FunctionName=xldeprecated  Parameters=nin,nout  mask(Xilinx Converter Block){arith_type=Signed  (2's comp), n_bits=8, bin_pt=6, quantization=Truncate, overflow=Wrap, latency=0, explicit_period=off, period=1, dbl_ovrd=off, show_param=off, inserted_by_tool=off, pipeline=off, xl_area=[0, 0, 0, 0, 0, 0, 0], xl_use_area=off}
      mask prompts: arith_type "Output Type"; n_bits "Number of Bits"; bin_pt "Binary Point"; quantization "Quantization Behavior"; overflow "Overflow Behavior"; explicit_period "Use Explicit Sample Period"; period "Sample Period"; dbl_ovrd "Override with Doubles"; show_param "---------------------- Show Implementation Parameters -----------------------------------------------------------------------------------"; inserted_by_tool "Hidden Parameter:  inserted_by_tool"; pipeline "Pipeline to Greatest Extent Possible"; xl_area "FPGA Area [Slices, FFs, BRAMs, LUTs, IOBs, Emb. Mults, TBUFs]"; xl_use_area "Use Area Above For Estimation"
      mask help:
      | BLOCK IS OUT OF DATE.
      |
      | This block is from an outdated copy of the Xilinx Blockset. Please run xlUpdateModel('<model-name>') to update to the latest version.
      mask init:
      | [designRoot, family, part, speed, package, simulinkPeriod, sysclkPeriod, dbl_ovrd, trimVbit] = xlSysgenSettings(gcb,1,1);
      | if (arith_type==1)
      |   bool = 1;
      | else
      |   bool = 0;
      |   arith_type = arith_type-1;
      | end
      | zstr=''; zpstr='';
      | if latency > 0
      |   zstr = 'z';
      |   zpstr = sprintf('-%d', latency);
      | end
      | [bg,fg] = xlcmap_r3('XBlock',dbl_ovrd);
      | if (inserted_by_tool)
      |   bg = [1.00 0.50 0.25];
      | end
      | iPos = get_param(gcb,'Position');
      | iWidth=iPos(3)-iPos(1); iHeight=iPos(4)-iPos(2);
      | iCx=iWidth/2;
      | iCy=iHeight/2;
      | [logoX, logoY] = xlogo(iPos);
      | zstrx = 0.45*iWidth-11; if (zstrx<3) zstrx=3; end
      | zstry = 0.36*iHeight-7; if (zstry<3) zstry=3; end
      | 
      | 
      | % one time added for param list
      | dblOvrd = dbl_ovrd;
      | precision0 = 2;
      | z0 = [n_bits bin_pt arith_type quantization overflow];
      | explicitClk = explicit_period;
      | 
      | 
      | % just pass everything to s-function
      | sfcn_mwsv__ = get_param(gcb, 'MaskWSVariables');
      | 
      | nport = get_param(gcbh, 'ports');
      | nin = nport(1);
      | nout = nport(2);
      mask Help: eval('xlWeb(xlhtmldoclink(''Convert''))');
      mask StyleString: popup(Boolean|Unsigned|Signed  (2's comp)),edit,edit,popup(Truncate|Round  (unbiased: +/- Inf)|Round  (unbiased: Even Values)),popup(Wrap|Saturate|Error),edit,checkbox,edit,checkbox,checkbox,checkbox,checkbox,edit,checkbox
      mask Display:
      | patch([0 iWidth iWidth 0],[0 0 iHeight iHeight] , bg);
      | patch(logoX,logoY , fg);
      | text(zstrx,zstry,zstr);
      | text(zstrx+5,zstry+5,zpstr);
      | port_label('output',1,'cast');
      | plot([0 0 iWidth iWidth 0], [0 iHeight iHeight 0 0]);
  Convolutional Encoder : S-Function  FunctionName=xldeprecated  Parameters=nin,nout  mask(Xilinx Convolutional Encoder){clength=3, conv_codes=[7 5 6], explicit_period=off, period=1, rst=off, en=off, dbl_ovrd=off, show_param=off, use_rpm=on, gen_core=off, xl_area=[0, 0, 0, 0, 0, 0, 0], xl_use_area=off}
      mask prompts: clength "Constraint Length"; conv_codes "Convolution Code Array (octal)"; explicit_period "Use Explicit Sample Period"; period "Sample Period  (use -1 to inherit first known input period)"; rst "Provide Reset Port"; en "Provide Enable Port"; dbl_ovrd "Override with Doubles"; show_param "---------------------- Show Implementation Parameters -----------------------------------------------------------------------------------"; use_rpm "Use Placement Information for Core"; gen_core "Generate Core"; xl_area "FPGA Area [Slices, FFs, BRAMs, LUTs, IOBs, Emb. Mults, TBUFs]"; xl_use_area "Use Area Above For Estimation"
      mask help:
      | BLOCK IS OUT OF DATE.
      |
      | This block is from an outdated copy of the Xilinx Blockset. Please run xlUpdateModel('<model-name>') to update to the latest version.
      mask init:
      | numstr3 = 2;
      | numstr4 = 2;
      | numstr5 = 2;
      | numstr6 = 2;
      | numstr7 = 2;
      | outstr3 = ''; outstr4 = ''; outstr5 = ''; outstr6 = ''; outstr7 = '';
      | [enPortNum,enPortStr,rstPortNum,rstPortStr] = xlport_en_rst(en,rst,3);
      | code_struct = xlconvertcodes(clength,conv_codes);
      | output_rate = code_struct.output_rate;
      | voutport = output_rate+1;
      | ccsucc = code_struct.success;
      | ccerror = code_struct.errorCode;
      | for i=1:output_rate,
      |   eval(sprintf('ccode%d = code_struct.code%d;',i,i));
      | end
      | for j=3:output_rate,
      |  eval(sprintf('numstr%d = %d;',j,j));
      |  eval(sprintf('outstr%d = ''dout%d'';',j,j));
      | end
      | [designRoot, family, part, speed, package, simulinkPeriod, sysclkPeriod, dbl_ovrd, trimVbit] = xlSysgenSettings(gcb,1,0);
      | trimVbit=1;
      | [bg,fg] = xlcmap_r3('XBlock',dbl_ovrd);
      | iPos = get_param(gcb,'Position');
      | iWidth=iPos(3)-iPos(1); iHeight=iPos(4)-iPos(2);
      | iCx=iWidth/2;
      | iCy=iHeight/2;
      | [logoX, logoY] = xlogo(iPos);
      | str = sprintf('Encoder Rate\n 1/%d',output_rate);
      | % one time added for param list
      | orate = output_rate;
      | latency = 1;
      | dblOvrd = dbl_ovrd;
      | useCore = 1;
      | precision0 = 1;
      | precision1 = 1; precision2 = 1;
      | precision3 = 1;
      | precision4 = 1;
      | precision5 = 1;
      | precision6 = 1;
      | precision7 = 1;
      | explicitClk = explicit_period;
      | rpm = use_rpm;
      | hasEN = en;
      | hasRST = rst;
      | gen_core = 1;
      | % just pass everything to s-function
      | sfcn_mwsv__ = get_param(gcb, 'MaskWSVariables');
      | 
      | nport = get_param(gcbh, 'ports');
      | nin = nport(1);
      | nout = nport(2);
      mask Help: eval('xlWeb(xlhtmldoclink(''Convolutional Encoder''))');
      mask Display:
      | patch([0 iWidth iWidth 0],[0 0 iHeight iHeight] , bg);
      | patch(logoX,logoY , fg);
      | port_label('input',1,'din');
      | port_label('output',1,'dout1' );
      | port_label('output',2,'dout2');
      | port_label('output',numstr3,outstr3);
      | port_label('output',numstr4,outstr4);
      | port_label('output',numstr5,outstr5);
      | port_label('output',numstr6,outstr6);
      | port_label('output',numstr7,outstr7);
      | port_label('output',voutport,'vout');
      | port_label('input',enPortNum,enPortStr);
      | port_label('input',rstPortNum,rstPortStr);
      | port_label('input',2,'vin');
      | plot([0 0 iWidth iWidth 0], [0 iHeight iHeight 0 0]);
  Counter : S-Function  FunctionName=xldeprecated  Parameters=nin,nout  mask(Xilinx Counter Block){cnt_type=Count Limited, n_bits=8, bin_pt=0, arith_type=Signed  (2's comp), start_count=0, cnt_to=Inf, cnt_by_val=1, operation=Up, explicit_period=off, period=1, load_pin=off, rst=off, en=off, dbl_ovrd=off, show_param=off, use_rpm=on, gen_core=off, xl_area=[0, 0, 0, 0, 0, 0, 0], xl_use_area=off}
      mask prompts: cnt_type "Counter Type"; n_bits "Number of Bits"; bin_pt "Binary Point Position"; arith_type "Arithmetic Type"; start_count "Initial Value"; cnt_to "Count To Value"; cnt_by_val "Step"; operation "Count Direction"; explicit_period "Use Explicit Sample Period"; period "Sample Period"; load_pin "Provide Load Port"; rst "Provide Reset Port"; en "Provide Enable Port"; dbl_ovrd "Override with Doubles"; show_param "---------------------- Show Implementation Parameters -----------------------------------------------------------------------------------"; use_rpm "Use Placement Information for Core"; gen_core "Generate Core"; xl_area "FPGA Area [Slices, FFs, BRAMs, LUTs, IOBs, Emb. Mults, TBUFs]"; xl_use_area "Use Area Above For Estimation"
      mask help:
      | BLOCK IS OUT OF DATE.
      |
      | This block is from an outdated copy of the Xilinx Blockset. Please run xlUpdateModel('<model-name>') to update to the latest version.
      mask init:
      | if ((rst==1) | (en==1) | (operation == 3) | ( (cnt_type == 2)&(load_pin == 1)))
      |   explicitClk = explicit_period;
      | else
      |   explicitClk =1;
      | end
      | numinputs = 0;
      | upDir = 'output';
      | upPNum = 1;
      | upStr = '';
      | loadDir = 'output';
      | loadPNum = 1;
      | loadStr = '';
      | dinDir = 'output';
      | dinPNum = 1;
      | dinStr = '';
      | if (operation == 3)
      |    numinputs = numinputs + 1;
      |    upDir = 'input';
      |   upPNum = numinputs;
      |    upStr = 'up';
      | end
      | 
      | if (cnt_type == 2)
      |   if (load_pin)
      |     loadDir = 'input';
      |     loadStr = 'load';
      |     numinputs = numinputs + 1;
      |     loadPNum = numinputs;
      |     dinDir = 'input';
      |     dinStr = 'din';
      |     numinputs = numinputs + 1;
      |     dinPNum = numinputs;
      |  end
      | end
      | numinputs = numinputs + 1;
      | [designRoot, family, part, speed, package, simulinkPeriod, sysclkPeriod, dbl_ovrd, trimVbit] = xlSysgenSettings(gcb,1,1);
      | [enPortNum, enPortStr, rstPortNum, rstPortStr, portDir] = xlport_en_rst(en, rst, numinputs);
      | [bg,fg]=xlcmap_r3('XBlock',dbl_ovrd);
      | iPos = get_param(gcb,'Position');
      | iWidth=iPos(3)-iPos(1); iHeight=iPos(4)-iPos(2);
      | iCx=iWidth/2;
      | iCy=iHeight/2;
      | [logoX, logoY] = xlogo(iPos);
      | 
      | 
      | % one time added for param list
      | dblOvrd = dbl_ovrd;
      | precision0 = 2;
      | z0 = [n_bits bin_pt arith_type  1 1];
      | hasEN = en;
      | hasRST = rst;
      | hasLoad = load_pin;
      | latency = 1;
      | useCore = 1;
      | gen_core = 1;
      | 
      | % just pass everything to s-function
      | sfcn_mwsv__ = get_param(gcb, 'MaskWSVariables');
      | nport = get_param(gcbh, 'ports');
      | nin = nport(1);
      | nout = nport(2);
      mask Help: eval('xlWeb(xlhtmldoclink(''Counter''))');
      mask StyleString: popup(Count Limited|Free Running),edit,edit,popup(Unsigned|Signed  (2's comp)),edit,edit,edit,popup(Up|Down|Up/Down),checkbox,edit,checkbox,checkbox,checkbox,checkbox,checkbox,checkbox,checkbox,edit,checkbox
      mask Display:
      | patch([0 iWidth iWidth 0],[0 0 iHeight iHeight] , bg);
      | patch(logoX,logoY , fg);
      | port_label('output',1,'out');
      | port_label(upDir,upPNum,upStr);
      | port_label(dinDir,dinPNum,dinStr);
      | port_label(loadDir,loadPNum,loadStr);
      | port_label(portDir,rstPortNum,rstPortStr);
      | port_label(portDir,enPortNum,enPortStr);
      | plot([0 0 iWidth iWidth 0], [0 iHeight iHeight 0 0]);
  DDS : S-Function  Description=Direct Digital Synthesizer  FunctionName=xldeprecated  Parameters=nin,nout  mask(Xilinx Direct Digital Synthesizer){mode=Sine and Cosine, n_bits=32, show_phase_param=off, phase_increment_type=Constant, phase_increment=1/10, phase_offset_type=None, phase_offset=1/4, show_internal_param=off, lut_addr_bits=10, acc_latency=One Cycle, acc_n_bits=32, phase_dithering=off, explicit_period=off, period=1, rst=off, en=on, dbl_ovrd=off, show_params=off, mem_type=Distributed Memory, pipeline=on, use_rpm=on, gen_core=off, xl_area=[0, 0, 0, 0, 0, 0, 0], xl_use_area=off}
      mask prompts: mode "Function"; n_bits "Output Width"; show_phase_param "---------------------- Show Phase Increment and Offset Parameters --------------------------------------------"; phase_increment_type "Phase Increment Type"; phase_increment "Normalized Phase Increment  (cycles per sample)"; phase_offset_type "Phase Offset Type"; phase_offset "Normalized Phase Offset  (cycles per sample)"; show_internal_param "---------------------- Show Configuration Parameters -----------------------------------"; lut_addr_bits "Lookup Table Input Width"; acc_latency "Accumulator Latency"; acc_n_bits "Accumulator Width"; phase_dithering "Use Phase Dithering"; explicit_period "Use Explicit Sample Period"; period "Sample Period"; rst "Provide Reset Port"; en "Provide Enable Port"; dbl_ovrd "Override with Doubles"; show_params "---------------------- Show Implementation Parameters ------------------------------------"; mem_type "Memory Type"; pipeline "Pipeline to Greatest Extent Possible"; use_rpm "Use Placement Information for Core"; gen_core "Generate Core"; xl_area "FPGA Area [Slices, FFs, BRAMs, LUTs, IOBs, Emb. Mults, TBUFs]"; xl_use_area "Use Area Above For Estimation"
      mask help:
      | BLOCK IS OUT OF DATE.
      |
      | This block is from an outdated copy of the Xilinx Blockset. Please run xlUpdateModel('<model-name>') to update to the latest version.
      mask init:
      | pitype = phase_increment_type;
      | potype = phase_offset_type;
      | mdata = 1;inp1= '';
      | mwe = 1;inp2= '';
      | ma = 1;  inp3= '';
      | portstr = 'output';
      | if (mode==1| mode == 5|mode==7)
      |   sstr = 'sin';
      |  else
      |   sstr = '-sin';
      | end
      | if (mode==3 | mode == 5 | mode == 6)
      |   cstr = 'cos';
      |  else
      |    cstr = '-cos';
      | end
      | mprt=1; mstr='';ostr2='';
      | if (mode==1| mode == 2)  ostr=sstr; end;
      | if (mode==3 | mode == 4)  ostr=cstr; end;
      | if (mode>4)  mprt=2; ostr=sstr; ostr2=cstr; end;
      | 
      | if(potype==3 & pitype == 2)
      |   explicitClk = explicit_period;
      |   portstr = 'input';
      |    mdata = 1;
      |    inp1 = 'data';
      |   mwe = 2;
      |    inp2 = 'we';
      |   ma = 3;
      |   inp3 = 'select';
      |  [enPortNum,enPortStr,rstPortNum,rstPortStr,portDir] = xlport_en_rst(en,rst,4);
      | elseif((potype==3 & pitype ==1 ) | (pitype==2 & (potype ==1 | potype == 2) ))
      |   portstr = 'input';
      |   mdata = 1;
      |   inp1 = 'data';
      |   mwe = 2;
      |   inp2 = 'we';
      |   [enPortNum,enPortStr,rstPortNum,rstPortStr,portDir] = xlport_en_rst(en,rst,3);
      |   explicitClk = explicit_period;
      | else
      |  [enPortNum,enPortStr,rstPortNum,rstPortStr, portDir] = xlport_en_rst(en,rst,1);
      |  if(en == 0 & rst == 0)
      |      explicitClk = 1;
      |  else
      |      explicitClk = explicit_period;
      |  end
      | 
      | end
      | [bg,fg] = xlcmap_r3('XBlock',dbl_ovrd);
      | iPos = get_param(gcb,'Position');
      | iWidth=iPos(3)-iPos(1); iHeight=iPos(4)-iPos(2);
      | iCx=iWidth/2;
      | iCy=iHeight/2;
      | [logoX, logoY] = xlogo(iPos);
      | zstrx = 0.45*iWidth-3; if (zstrx<3) zstrx=3; end
      | zstry = 0.36*iHeight-7; if (zstry<3) zstry=3; end
      | % one time added for param list
      | [designRoot, family, part, speed, package, simulinkPeriod, sysclkPeriod, dbl_ovrd, trimVbit] = xlSysgenSettings(gcb,1,1);
      | bin_pt = n_bits-1;
      | phase_angle_width = lut_addr_bits;
      | pd = phase_dithering;
      | memtype = mem_type;
      | hasEN = en;
      | hasRST = rst;
      | accwidth = acc_n_bits;
      | phase_inc = phase_increment;
      | dblOvrd = dbl_ovrd;
      | precision0 = 2;
      | z0 = [n_bits bin_pt 2 2 2];
      | useCore = 1;
      | pipelined = pipeline;
      | precision1 = 2;
      | z1 = [n_bits bin_pt 2 2 2];
      | gen_core = 1;
      | 
      | % just pass everything to s-function
      | sfcn_mwsv__ = get_param(gcb, 'MaskWSVariables');
      | 
      | nport = get_param(gcbh, 'ports');
      | nin = nport(1);
      | nout = nport(2);
      mask Help: eval('xlWeb(xlhtmldoclink(''DDS''))');
      mask StyleString: popup(Sine|Negative Sine|Cosine|Negative Cosine|Sine and Cosine|Negative Sine and Cosine|Sine and Negative Cosine|Negative Sine and Negative Cosine),edit,checkbox,popup(Constant|Register),edit,popup(None|Constant|Register),edit,checkbox,edit,popup(Zero Cycle|One Cycle),edit,checkbox,checkbox,edit,checkbox,checkbox,checkbox,checkbox,popup(Distributed Memory|Block RAM),checkbox,checkbox,checkbox,edit,checkbox
      mask Display:
      | patch([0 iWidth iWidth 0],[0 0 iHeight iHeight] , bg);
      | patch(logoX,logoY , fg);
      | port_label('output',1,ostr);
      | port_label('output',mprt,ostr2);
      | port_label(portstr,mdata,inp1);
      | port_label(portstr,mwe,inp2);
      | port_label(portstr,ma,inp3);
      | port_label(portDir,enPortNum,enPortStr);
      | port_label(portDir,rstPortNum,rstPortStr);
      | ;plot([0 0 iWidth iWidth 0], [0 iHeight iHeight 0 0]);
  DSP48 : S-Function  FunctionName=xldeprecated  Parameters=nin,nout  mask(Xilinx DSP48){pipeline_a=1, use_b=Direct from B Port, pipeline_b=1, pipeline_bcin=0, pipeline_c=on, pipeline_p=on, pipeline_mult=on, pipeline_opmode=on, pipeline_sub=on, pipeline_carryin=on, pipeline_carryinsel=on, use_op=off, use_creg=off, use_pcin=off, use_pcout=off, use_bcout=off, access_rst=off, rst_all=off, rst_a=off, rst_b=off, rst_bcin=off, rst_c=off, rst_mult=off, rst_p=off, rst_ctrl=off, rst_carry_in=off, access_en=off, en_all=off, en_a=off, en_b=off, en_bcin=off, en_c=off, en_mult=off, en_p=off, en_carry_in=off, en_ctrl=off, explicit_period=off, period=1, dbl_ovrd=off, show_param=off, xl_useadderonly=off, xl_area=[0, 0, 0, 0, 0, 0, 0], xl_use_area=off}
      mask prompts: pipeline_a "Length of A Pipeline"; use_b "B Input"; pipeline_b "Length of B Pipeline"; pipeline_bcin "Length of BCIN Pipeline"; pipeline_c "Pipeline Input C"; pipeline_p "Pipeline P"; pipeline_mult "Pipeline Multiplier"; pipeline_opmode "Pipeline OpMode"; pipeline_sub "Pipeline Subtract"; pipeline_carryin "Pipeline Carry In"; pipeline_carryinsel "Pipeline Carry In Sel"; use_op "Consolidate Control Port (opmode, subtract, carry_in, carry_in_sel)"; use_creg "Provide C Port"; use_pcin "Provide PCIN Port"; use_pcout "Provide PCOUT Port"; use_bcout "Provide BCOUT Port"; access_rst "---------------------- Access Reset Port Controls ---------------------------------------------------------"; rst_all "Provide Global Reset Port"; rst_a "Provide Reset Port for A"; rst_b "Provide Reset Port for B"; rst_bcin "Provide Reset Port for BCIN"; rst_c "Provide Reset Port for C"; rst_mult "Provide Reset Port for Multiplier"; rst_p "Provide Reset Port for P"; rst_ctrl "Provide Reset Port for Controls (Subtract, CarryInSel, OpMode)"; rst_carry_in "Provide Reset Port for Carry In"; access_en "---------------------- Access Enable Port Controls ---------------------------------------------------------"; en_all "Provide Global Enable Port"; en_a "Provide Enable Port for A"; en_b "Provide Enable Port for B"; en_bcin "Provide Enable Port for BCIN"; en_c "Provide Enable Port for C"; en_mult "Provide Enable Port for Multiplier"; en_p "Provide Enable Port for P"; en_carry_in "Provide Enable Port for Carry In"; en_ctrl "Provide Enable Port for Controls (Subtract, CarryInSel, OpMode)"; explicit_period "Use Explicit Sample Period"; period "Sample Period  (use -1 to inherit first known input period)"; dbl_ovrd "Override with Doubles"; show_param "---------------------- Show Implementation Parameters -----------------------------------------------------------------------------------"; xl_useadderonly "Use Adder Only"; xl_area "FPGA Area [Slices, FFs, BRAMs, LUTs, IOBs, Emb. Mults, TBUFs]"; xl_use_area "Use Area Above For Estimation"
      mask help:
      | BLOCK IS OUT OF DATE.
      |
      | This block is from an outdated copy of the Xilinx Blockset. Please run xlUpdateModel('<model-name>') to update to the latest version.
      mask init:
      | [designRoot, family, part, speed, package, simulinkPeriod, sysclkPeriod, dbl_ovrd, trimVbit] = xlSysgenSettings(gcb,1,0);
      | trimVbit=1;
      | [bg,fg] = xlcmap_r3('XBlock',dbl_ovrd);
      | iPos = get_param(gcb,'Position');
      | iWidth=iPos(3)-iPos(1); iHeight=iPos(4)-iPos(2);
      | iCx=iWidth/2;
      | iCy=iHeight/2;
      | [logoX, logoY] = xlogo(iPos);
      | opt_ports = 3; % default starting port num for optional ports
      | %initialize all the strings
      | b_str = 'a'; b_num = 1;
      | c_str = 'a'; c_num = 1;
      | ce_all_str = 'a'; rst_all_str = 'a';
      | ce_a_str = 'a'; rst_a_str = 'a';
      | ce_b_str = 'a'; rst_b_str = 'a';
      | ce_c_str = 'a'; rst_c_str = 'a';
      | ce_mult_str = 'a'; rst_mult_str = 'a';
      | ce_p_str = 'a'; rst_p_str = 'a';
      | ce_ctrl_str = 'a'; rst_ctrl_str = 'a';
      | ce_carryin_str = 'a'; rst_carryin_str = 'a';
      | ce_cinsub_str = 'a'; rst_cinsub_str = 'a';
      | bcin_str = 'a'; pcin_str = 'a';
      | pcout_str = 'p'; bcout_str = 'p';
      | opstr = 'a'; sub_str = 'a'; carryin_str = 'a';
      | carryin_sel_str = 'a';
      | % initialize all the port nums
      | ce_all_num = 1; rst_all_num = 1;
      | ce_a_num = 1; rst_a_num = 1;
      | ce_b_num = 1; rst_b_num = 1;
      | ce_c_num = 1; rst_c_num = 1;
      | ce_p_num = 1; rst_p_num = 1;
      | ce_mult_num = 1; rst_mult_num = 1;
      | ce_ctrl_num = 1; rst_ctrl_num = 1;
      | ce_carryin_num = 1; rst_carryin_num = 1;
      | ce_cinsub_num = 1; rst_cinsub_num = 1;
      | bcin_num = 1; pcin_num = 1;
      | pcout_num = 1; bcout_num = 1;
      | opnum = 1; sub_num = 1;
      | carryin_num = 1; carryin_sel_num = 1;
      | %Determine output ports
      | if(use_bcout == 1)
      | 	bcout_num = 2;
      | 	bcout_str = 'bcout';
      | end
      | if(use_pcout == 1)
      | 	if(use_bcout == 1)
      | 		pcout_num = 3;
      | 	else
      | 		pcout_num = 2;
      | 	end
      | 	pcout_str = 'pcout';
      | end
      | %determine to use b or bcin
      | if(use_b == 1) % USE B
      | 	b_str = 'b';
      | 	b_num = 2;
      | end
      | if(use_b == 2) % USE BCIN - place in same location as B
      | 	bcin_num = 2;
      | 	bcin_str = 'bcin';
      | end
      | if(use_creg == 1)
      | 	c_num = 3;
      | 	opt_ports = 4;
      | 	c_str = 'c';
      | end
      | if(use_pcin == 1)
      | 	pcin_num = opt_ports;
      | 	pcin_str = 'pcin';
      | 	opt_ports = opt_ports + 1;
      | end
      | %determine to use consolidated opmode or not
      | if(use_op == 1)
      | 	opnum = opt_ports;
      | 	opt_ports = opt_ports + 1;
      | 	opstr = 'op';
      | else
      | 	opnum = opt_ports;
      | 	opstr = 'opmode';
      | 	opt_ports = opt_ports + 1;
      | 	sub_num = opt_ports;
      | 	sub_str = 'subtract';
      | 	opt_ports = opt_ports + 1;
      | 	carryin_num = opt_ports;
      | 	carryin_str = 'carry_in';
      | 	opt_ports = opt_ports + 1;
      | 	carryin_sel_num = opt_ports;
      | 	carryin_sel_str = 'carry_in_sel';
      | 	opt_ports = opt_ports + 1;
      | end
      | %determine which optional ports to display
      | if(en_all == 1)
      | 	ce_a_str = 'en';
      | 	ce_a_num = opt_ports;
      | 	opt_ports = opt_ports + 1;
      | end
      | if(pipeline_a ~= 1 & en_a == 1 & en_all == 0)
      | 	ce_a_str = 'ce_a';
      | 	ce_a_num = opt_ports;
      | 	opt_ports = opt_ports + 1;
      | end
      | if(pipeline_b ~= 1 & (en_b == 1 || en_bcin == 1) & en_all == 0)
      | 	if(en_b == 1)
      | 		ce_b_str = 'ce_b';
      | 	end
      | 	if(en_bcin == 1)
      | 		ce_b_str = 'ce_bcin';
      | 	end
      | 	ce_b_num = opt_ports;
      | 	opt_ports = opt_ports + 1;
      | end
      | if(pipeline_c == 1 & en_c == 1 & en_all == 0)
      | 	ce_c_num = opt_ports;
      | 	ce_c_str = 'ce_c';
      | 	opt_ports = opt_ports + 1;
      | end
      | if(pipeline_mult == 1 & en_mult == 1 & en_all == 0)
      | 	ce_mult_num = opt_ports;
      | 	ce_mult_str = 'ce_m';
      | 	opt_ports = opt_ports + 1;
      | end
      | if(pipeline_p == 1 & en_p == 1 & en_all == 0)
      | 	ce_p_num = opt_ports;
      | 	ce_p_str = 'ce_p';
      | 	opt_ports = opt_ports + 1;
      | end	
      | if(en_ctrl == 1 & en_all == 0)
      | 	ce_ctrl_str = 'ce_ctrl';
      | 	ce_ctrl_num = opt_ports;
      | 	opt_ports = opt_ports + 1;
      | end
      | if(en_carry_in == 1 & en_all == 0)
      | 	ce_carryin_num = opt_ports;
      | 	ce_carryin_str = 'ce_carry_in';
      | 	opt_ports = opt_ports + 1;
      | end
      | if(en_ctrl == 1 & en_all == 0)
      | 	ce_cinsub_str = 'ce_cinsub';
      | 	ce_cinsub_num = opt_ports;
      | 	opt_ports = opt_ports + 1;
      | end
      | %determine which rst ports to display
      | if(rst_all == 1)
      | 	rst_a_str = 'rst';
      | 	rst_a_num = opt_ports;
      | 	opt_ports = opt_ports + 1;
      | end
      | if(pipeline_a ~= 1 & rst_a == 1 & rst_all == 0)
      | 	rst_a_str = 'rst_a';
      | 	rst_a_num = opt_ports;
      | 	opt_ports = opt_ports + 1;
      | end
      | if(pipeline_b ~= 1 & (rst_b == 1|| rst_bcin) & rst_all == 0)
      | 	if(rst_b == 1)
      | 		rst_b_str = 'rst_b';
      | 	end
      | 	if(rst_bcin == 1)
      | 		rst_b_str = 'rst_bcin';
      | 	end
      | 	rst_b_num = opt_ports;
      | 	opt_ports = opt_ports + 1;
      | end
      | if(pipeline_c == 1 & rst_c == 1 & rst_all == 0)
      | 	rst_c_num = opt_ports;
      | 	rst_c_str = 'rst_c';
      | 	opt_ports = opt_ports + 1;
      | end
      | if(pipeline_mult == 1 & rst_mult == 1 & rst_all == 0)
      | 	rst_mult_num = opt_ports;
      | 	rst_mult_str = 'rst_m';
      | 	opt_ports = opt_ports + 1;
      | end
      | if(pipeline_p == 1 & rst_p == 1 & rst_all == 0)
      | 	rst_p_num = opt_ports;
      | 	rst_p_str = 'rst_p';
      | 	opt_ports = opt_ports + 1;
      | end
      | if(rst_ctrl == 1 & rst_all == 0)
      | 	rst_ctrl_str = 'rst_ctrl';
      | 	rst_ctrl_num = opt_ports;
      | 	opt_ports = opt_ports + 1;
      | end
      | if(rst_carry_in == 1 & rst_all == 0) 
      | rst_carryin_num = opt_ports;
      | rst_carryin_str = 'rst_carry_in';
      | opt_ports = opt_ports + 1;
      | end
      | 
      | % one time added for param list
      | latency = 1;
      | dblOvrd = dbl_ovrd;
      | precision0 = 1;
      | precision1 = 1;
      | precision2 = 1;
      | precision3 = 1;
      | precision4 = 1;
      | precision5 = 1;
      | precision6 = 1;
      | precision7 = 1;
      | precision8 = 1;
      | precision9 = 1;
      | precision10 = 1;
      | precision11 = 1;
      | precision12 = 1;
      | precision13 = 1;
      | precision14 = 1;
      | precision15 = 1;
      | precision16 = 1;
      | precision17 = 1;
      | precision18 = 1;
      | precision19 = 1;
      | precision20 = 1;
      | precision21 = 1;
      | precision22 = 1;
      | precision23 = 1;
      | precision24 = 1;
      | precision25 = 1;
      | precision26 = 1;
      | explicitClk = explicit_period;
      | hasEN = 0;
      | hasRST = 0;
      | % just pass everything to s-function
      | sfcn_mwsv__ = get_param(gcb, 'MaskWSVariables');
      | 
      | nport = get_param(gcbh, 'ports');
      | nin = nport(1);
      | nout = nport(2);
      mask Help: eval('xlWeb(xlhtmldoclink(''DSP48''))');
      mask StyleString: popup(0|1|2),popup(Direct from B Port|Cascaded from BCIN Port),popup(0|1|2),popup(0|1|2),checkbox,checkbox,checkbox,checkbox,checkbox,checkbox,checkbox,checkbox,checkbox,checkbox,checkbox,checkbox,checkbox,checkbox,checkbox,checkbox,checkbox,checkbox,checkbox,checkbox,checkbox,checkbox,checkbox,checkbox,checkbox,checkbox,checkbox,checkbox,checkbox,checkbox,checkbox,checkbox,checkbox,edit,checkbox,checkbox,checkbox,edit,checkbox
      mask Display:
      | patch([0 iWidth iWidth 0],[0 0 iHeight iHeight] , bg);
      | patch(logoX,logoY , fg);
      | port_label('input',1,'a');
      | port_label('input',b_num,b_str);
      | port_label('input',c_num,c_str);
      | port_label('input',opnum,opstr);
      | port_label('input',sub_num,sub_str);
      | port_label('input',carryin_num,carryin_str);
      | port_label('input',carryin_sel_num,carryin_sel_str);
      | port_label('input',ce_a_num,ce_a_str);
      | port_label('input',ce_b_num,ce_b_str);
      | port_label('input',ce_c_num,ce_c_str);
      | port_label('input',ce_mult_num,ce_mult_str);
      | port_label('input',ce_p_num,ce_p_str);
      | port_label('input',ce_ctrl_num,ce_ctrl_str);
      | port_label('input',ce_carryin_num,ce_carryin_str);
      | port_label('input',ce_cinsub_num,ce_cinsub_str);
      | port_label('input',rst_a_num,rst_a_str);
      | port_label('input',rst_b_num,rst_b_str);
      | port_label('input',rst_c_num,rst_c_str);
      | port_label('input',rst_mult_num,rst_mult_str);
      | port_label('input',rst_p_num,rst_p_str);
      | port_label('input',rst_ctrl_num,rst_ctrl_str);
      | port_label('input',rst_carryin_num,rst_carryin_str);
      | port_label('input',bcin_num,bcin_str);
      | port_label('input',pcin_num,pcin_str);
      | port_label('output',bcout_num,bcout_str );
      | port_label('output',pcout_num,pcout_str);
      | port_label('output',1,'p');
      | plot([0 0 iWidth iWidth 0], [0 iHeight iHeight 0 0]);
  DSP48 Macro : Subsystem  mask(DSP48 Macro){instrlist=|, n_bits_a=18, bin_pt_a=11, arith_type_a=Signed  (2's comp), portalist=coeff, n_bits_b=18, bin_pt_b=0, arith_type_b=Signed  (2's comp), portblist=datain;zero, n_bits_c=30, bin_pt_c=0, arith_type_c=Signed  (2's comp), portclist=result, dbl_ovrd=off, precision=User Defined, n_bits=16, bin_pt=2, arith_type=Signed  (2's comp), pcout=off, bcout=off, pipeline=Max Speed, mode=Multiplier, rst=off, en=off, synth_opt=on, custom_opt=[1,1,1,1,1,1,0,0,0,0], period=-1, xlBlockVersion=0, statestr=|}
      mask instrlist=|
      | p =p+coeff*zero
      | p=coeff*datain
      | p=coeff*datain + result
      mask statestr=|
      | |p =p+coeff*zero
      | p=coeff*datain
      | p=coeff*datain + result
      | |18|11|Signed  (2's comp)|coeff|18|0|Signed  (2's comp)|datain;zero  |30|0|Signed  (2's comp)|result|off|User Defined|16|2|Signed  (2's comp)|off|off|Max Speed|Multiplier|off|off|on|[1,1,1,1,1,1,0,0,0,0]|-1  |0
      mask prompts: instrlist "Instruction List"; n_bits_a "Number of Bits in A"; bin_pt_a "Binary Point  in A"; arith_type_a "Arithmetic Type A"; portalist "Inputs to Port A"; n_bits_b "Number of Bits in B"; bin_pt_b "Binary Point in B"; arith_type_b "Arithmetic Type B"; portblist "Inputs to Port B"; n_bits_c "Number of Bits in C"; bin_pt_c "Binary Point in C"; arith_type_c "Arithmetic Type C"; portclist "Inputs to port C"; dbl_ovrd "Override With Doubles"; precision "Output Type"; n_bits "Number of Output Bits"; bin_pt "Output Binary Point"; arith_type "Output Arithmetic Type"; pcout "Provide PCOUT"; bcout "Provide BCOUT"; pipeline "Pipeline Options"; custom_opt "custom_pipleine"; period "Sample Time"; xlBlockVersion "Sysgen Version"
      mask help: Facililtates the user of the DSP48 block as a dynamic operator.
      mask init:
      | this_gcb = gcb;
      | this_gcs = gcs;
      | [bg,fg] = xlcmap_r3('XBlock',dbl_ovrd);
      | iPos = get_param(gcb,'Position');
      | iWidth=iPos(3)-iPos(1); iHeight=iPos(4)-iPos(2);
      | iCx=iWidth/2;
      | iCy=iHeight/2;
      | [logoX, logoY] = xlogo(iPos);
      | 
      | if (~strcmp(bdroot(this_gcs),'xbsDSP_r3'))
      | set_param(this_gcb,'linkstatus','none');
      | %cflag = xlchecksameDSP48(this_gcb);
      | xlinitpaneDSP48(this_gcb);
      | end;
      settings: OpenFcn=modelName = get_param(bdroot, 'name');h = errordlg(sprintf(['This block is from an outdated copy of the Xilinx Blockset.\nPlease run xlUpdateModel(''' modelName ''') to update this design.']), 'Update Required');
      mask Help: eval('xlWeb(xlhtmldoclink(''DSP48 Macro''))');
      mask StyleString: edit,edit,edit,popup(Signed  (2's comp)|Unsigned),edit,edit,edit,popup(Signed  (2's comp)|Unsigned),edit,edit,edit,popup(Signed  (2's comp)|Unsigned),edit,checkbox,popup(Full|User Defined),edit,edit,popup(Signed  (2's comp)|Unsigned),checkbox,checkbox,popup(Max Speed|Min Area|Custom),popup(Adder|Multiplier),checkbox,checkbox,checkbox,edit,edit,edit,edit
      mask Display:
      | patch([0 iWidth iWidth 0],[0 0 iHeight iHeight] , bg);
      | patch(logoX,logoY , fg);
      | plot([0 0 iWidth iWidth 0], [0 iHeight iHeight 0 0]);
      | port_label('input',1,'Sel');
      | port_label('input',2,'coeff');
      | port_label('input',3,'zero');
      | port_label('input',4,'datain');
      | port_label('input',5,'result');
      | port_label('output',1,'P');
  Delay : S-Function  FunctionName=xldeprecated  Parameters=nin,nout  mask(Xilinx Delay Block){latency=1, reg_retiming=off, explicit_period=off, period=1, en=off, accept_only_valid=off, init_zero=on, dbl_ovrd=off, show_param=off, xl_area=[0, 0, 0, 0, 0, 0, 0], xl_use_area=off}
      mask prompts: reg_retiming "Enable Register Retiming"; explicit_period "Use Explicit Sample Period"; period "Sample Period  (use -1 to inherit first known input period)"; en "Provide Enable Port"; accept_only_valid "Shift In Only Valid Data"; init_zero "Initialize with Zeros (otherwise Invalid)"; dbl_ovrd "Override with Doubles"; show_param "---------------------- Show Implementation Parameters -----------------------------------------------------------------------------------"; xl_area "FPGA Area [Slices, FFs, BRAMs, LUTs, IOBs, Emb. Mults, TBUFs]"; xl_use_area "Use Area Above For Estimation"
      mask help:
      | BLOCK IS OUT OF DATE.
      |
      | This block is from an outdated copy of the Xilinx Blockset. Please run xlUpdateModel('<model-name>') to update to the latest version.
      mask init:
      | rst = 0;
      | [enPortNum,enPortStr,rstPortNum,rstPortStr] = xlport_en_rst(en,rst,2);
      | str = sprintf('-%d',latency);
      | [designRoot, family, part, speed, package, simulinkPeriod, sysclkPeriod, dbl_ovrd, trimVbit] = xlSysgenSettings(gcb,1,1);
      | [bg,fg] = xlcmap_r3('XBlock',dbl_ovrd);
      | iPos = get_param(gcb,'Position');
      | iWidth=iPos(3)-iPos(1); iHeight=iPos(4)-iPos(2);
      | iCx=iWidth/2;
      | iCy=iHeight/2;
      | [logoX, logoY] = xlogo(iPos);
      | 
      | 
      | % one time added for param list
      | dblOvrd = dbl_ovrd;
      | vOnly = accept_only_valid;
      | initZero = init_zero;
      | precision0 = 1;
      | z0 = [0 0 1 1 1];
      | explicitClk = explicit_period;
      | 
      | hasRST = rst;
      | hasEN = en;
      | % just pass everything to s-function
      | sfcn_mwsv__ = get_param(gcb, 'MaskWSVariables');
      | 
      | nport = get_param(gcbh, 'ports');
      | nin = nport(1);
      | nout = nport(2);
      mask Help: eval('xlWeb(xlhtmldoclink(''Delay''))');
      mask Display:
      | patch([0 iWidth iWidth 0],[0 0 iHeight iHeight] , bg);
      | patch(logoX,logoY , fg);
      | text(iCx-6,iCy,'z');
      | text(iCx,iCy+4,str);
      | port_label('input',enPortNum,enPortStr);
      | ;plot([0 0 iWidth iWidth 0], [0 iHeight iHeight 0 0]);
  Depuncture : S-Function  FunctionName=xldeprecated  Parameters=nin,nout  mask(Xilinx Depuncture Block){insert_char=[1 0 0], insert_string='100', explicit_period=off, period=1, dbl_ovrd=off}
      mask prompts: insert_char "Puncture Code"; insert_string "Symbol to Insert"; explicit_period "Use Explicit Sample Period"; period "Sample Period"; dbl_ovrd "Override with Doubles"
      mask help:
      | BLOCK IS OUT OF DATE.
      |
      | This block is from an outdated copy of the Xilinx Blockset. Please run xlUpdateModel('<model-name>') to update to the latest version.
      mask init:
      | if  ( find((insert_char~=1) & (insert_char~=0)))
      |     insert_code = 'error';
      | else
      | insert_code = char( (insert_char ~= 0) + 48 );
      | end;
      | [designRoot, family, part, speed, package, simulinkPeriod, sysclkPeriod, dbl_ovrd, trimVbit] = xlSysgenSettings(gcb,1,1);
      | dbl_ovrdStr = '';
      | [bg,fg]=xlcmap_r3('XBlock',dbl_ovrd);
      | iPos = get_param(gcb,'Position');
      | iWidth=iPos(3)-iPos(1); iHeight=iPos(4)-iPos(2);
      | iCx=iWidth/2;
      | iCy=iHeight/2;
      | [logoX, logoY] = xlogo(iPos);
      | 
      | 
      | % one time added for param list
      | insert_int = bin2dec(insert_code);
      | string_int = bin2dec(insert_string);
      | dblOvrd = dbl_ovrd;
      | precision0 = 1;
      | explicitClk = explicit_period;
      | 
      | 
      | % just pass everything to s-function
      | sfcn_mwsv__ = get_param(gcb, 'MaskWSVariables');
      | 
      | nport = get_param(gcbh, 'ports');
      | nin = nport(1);
      | nout = nport(2);
      mask Help: eval('xlWeb(xlhtmldoclink(''Depuncture''))');
      mask Display:
      | patch([0 iWidth iWidth 0],[0 0 iHeight iHeight] , bg);
      | patch(logoX,logoY , fg);
      | port_label('output',1,'Depuncture');
      | 
      | ;plot([0 0 iWidth iWidth 0], [0 iHeight iHeight 0 0]);
  Digital Up Converter : S-Function  FunctionName=xldeprecated  Parameters=nin,nout  mask(Digital Up Converter){}
      mask help:
      | BLOCK IS OUT OF DATE.
      |
      | This block is from an outdated copy of the Xilinx Blockset. Please run xlUpdateModel('<model-name>') to update to the latest version.
      mask init:
      | % Set Block Logo
      | [bg,fg] = xlcmap_r3('XBlock',0);
      | iPos = get_param(gcb,'Position');
      | iWidth=iPos(3)-iPos(1); iHeight=iPos(4)-iPos(2);
      | iCx=iWidth/2;
      | iCy=iHeight/2;
      | [logoX, logoY] = xlogo(iPos);
      | 
      | errormsg = ['This block has not yet been installed.  You may download this and other blocks from the Xilinx web site by clicking on the block help button.'];
      | num_inports = 0;
      | num_outports = 0;
      | nport = get_param(gcbh, 'ports');
      | nin = nport(1);
      | nout = nport(2);
      mask Help: eval('xlWeb(xlhtmldoclink(''Digital Up Converter''))');
      mask Display:
      | patch([0 iWidth iWidth 0],[0 0 iHeight iHeight] , bg);
      | patch(logoX,logoY, fg);
      | text(iCx-29,iCy,'Not Installed');
      | plot([0 0 iWidth iWidth 0], [0 iHeight iHeight 0 0]);
  Disregard Subsystem : Subsystem  Tag=discardX  mask(Xilinx Disregard Subsystem For Generation){}
      mask help: Place this block into any subsystem of a model to indicate that you do not wish System Generator to generate any hardware components for the subsystem. This block can be used in combination with the Simulation Multiplexer block to build alternative simulation models for a portion of a design (e.g. to provide a simulation model for a black box).
      mask init:
      | [bg,fg]=xlcmap_r3('BlkBox');
      | iPos = get_param(gcb,'Position');
      | iWidth=iPos(3)-iPos(1); iHeight=iPos(4)-iPos(2);
      | iCx=iWidth/2;
      | iCy=iHeight/2;
      | [logoX, logoY] = xlogo(iPos);
      settings: AttributesFormatString=Disregard Subsystem\nFor Generation  OpenFcn=modelName = get_param(bdroot, 'name');h = errordlg(sprintf(['This block is from an outdated copy of the Xilinx Blockset.\nPlease run xlUpdateModel(''' modelName ''') to update this design.']), 'Update Required');
      mask Help: eval('xlWeb(xlhtmldoclink(''Disregard Subsystem''))');
      mask Display:
      | patch([0 iWidth iWidth 0],[0 0 iHeight iHeight] , bg);
      | patch(logoX,logoY, fg);
      | ;plot([0 0 iWidth iWidth 0], [0 iHeight iHeight 0 0]);
  Down Sample : S-Function  FunctionName=xldeprecated  Parameters=nin,nout  mask(Xilinx Down Sampling Block){sample_ratio=2, sample_phase=Last Value of Frame  (most efficient), latency=1, en=off, dbl_ovrd=off, show_param=off, xl_area=[0, 0, 0, 0, 0, 0, 0], xl_use_area=off}
      mask prompts: sample_ratio "Sampling Rate (number of input samples per output sample)"; sample_phase "Sample"; en "Provide Enable Port"; dbl_ovrd "Override with Doubles"; show_param "---------------------- Show Implementation Parameters -----------------------------------------------------------------------------------"; xl_area "FPGA Area [Slices, FFs, BRAMs, LUTs, IOBs, Emb. Mults, TBUFs]"; xl_use_area "Use Area Above For Estimation"
      mask help:
      | BLOCK IS OUT OF DATE.
      |
      | This block is from an outdated copy of the Xilinx Blockset. Please run xlUpdateModel('<model-name>') to update to the latest version.
      mask init:
      | % get enable port number and string
      | [enPortNum, enPortStr] =xlport_en_rst(en,0,2);
      | 
      | zstr='';
      | zpstr='';
      | if latency > 0
      |   zstr = 'z';
      |   zpstr = sprintf('-%d', latency);
      | end
      | 
      | str = sprintf(' %d',floor(sample_ratio));
      | [designRoot, family, part, speed, package, simulinkPeriod, sysclkPeriod, dbl_ovrd, trimVbit] = xlSysgenSettings(gcb,1,1);
      | [bg,fg] = xlcmap_r3('XBlock',dbl_ovrd);
      | iPos = get_param(gcb,'Position');
      | iWidth=iPos(3)-iPos(1); iHeight=iPos(4)-iPos(2);
      | iCx=iWidth/2;
      | iCy=iHeight/2;
      | [logoX, logoY] = xlogo(iPos);
      | aw = 3;
      | ah = 7;
      | arrowX = [0 (-aw) (-aw) 0 0 (1) (1) (aw+1) (aw+1) (1)];
      | arrowY = [(ah-1) (ah-aw-1) (ah-aw) (ah) (-ah) (-ah) (ah) (ah-aw) (ah-aw-1) (ah-1)];
      | arrowX = arrowX + iCx - 2 - 3.5*length(str);
      | arrowY = iCy - arrowY + 2;
      | zstrx = 0.45*iWidth-3; if (zstrx<3) zstrx=3; end
      | zstry = 0.36*iHeight-7; if (zstry<3) zstry=3; end
      | 
      | % one time added for param list
      | precision0 = 1;
      | dblOvrd = dbl_ovrd;
      | ratio = sample_ratio;
      | samplePhase = sample_phase;
      | hasEN = en;
      | 
      | 
      | % just pass everything to s-function
      | sfcn_mwsv__ = get_param(gcb, 'MaskWSVariables');
      | 
      | nport = get_param(gcbh, 'ports');
      | nin = nport(1);
      | nout = nport(2);
      mask Help: eval('xlWeb(xlhtmldoclink(''Down Sample''))');
      mask StyleString: edit,popup(First Value of Frame|Last Value of Frame  (most efficient)),edit,checkbox,checkbox,checkbox,edit,checkbox
      mask Display:
      | patch([0 iWidth iWidth 0],[0 0 iHeight iHeight] , bg);
      | patch(logoX,logoY , fg);
      | plot(arrowX,arrowY);
      | disp(str);
      | text(zstrx,zstry,zstr);
      | text(zstrx+5,zstry+5,zpstr);
      | port_label('input',enPortNum,enPortStr);
      | 
      | ;plot([0 0 iWidth iWidth 0], [0 iHeight iHeight 0 0]);
  Dual Port RAM : S-Function  FunctionName=xldeprecated  Parameters=nin,nout  mask(Xilinx Dual Port Random Access Memory){depth=16, initVector=sin(pi*(0:15)/16), write_mode_A=Read After Write, write_mode_B=Read After Write, latency=1, mem_collision=off, init_zero=on, explicit_period=off, period=1, dbl_ovrd=off, rst_a=off, init_a=0, rst_b=off, init_b=0, show_param=off, distributed_mem=off, use_rpm=off, gen_core=off, xl_area=[0, 0, 0, 0, 0, 0, 0], xl_use_area=off}
      mask prompts: initVector "Initial Value Vector"; write_mode_A "Write Mode:  Port A"; write_mode_B "Write Mode:  Port B"; mem_collision "Provide Output Valid Port"; init_zero "Zero Initial Output  (otherwise NaN)"; explicit_period "Use Explicit Sample Period"; period "Sample Period  (use -1 to inherit first known input period)"; dbl_ovrd "Override with Doubles"; rst_a "Provide Reset Port for Port A Output Register"; init_a "Initial Value for Port A Output Register"; rst_b "Provide Reset Port for Port B Output Register"; init_b "Initial Value for Port B Output Register"; show_param "---------------------- Show Implementation Parameters -----------------------------------------------------------------------------------"; distributed_mem "Use Distributed Memory (instead of block RAM)"; use_rpm "Use Placement Information for Core"; gen_core "Generate Core"; xl_area "FPGA Area [Slices, FFs, BRAMs, LUTs, IOBs, Emb. Mults, TBUFs]"; xl_use_area "Use Area Above For Estimation"
      mask help:
      | BLOCK IS OUT OF DATE.
      |
      | This block is from an outdated copy of the Xilinx Blockset. Please run xlUpdateModel('<model-name>') to update to the latest version.
      mask init:
      | [designRoot, family, part, speed, package, simulinkPeriod, sysclkPeriod, dbl_ovrd, trimVbit] = xlSysgenSettings(gcb,1,1);
      | if isempty(family)
      | 	family = 'Virtex2';
      | end;
      | dbl_ovrdStr = '';
      | [bg,fg] = xlcmap_r3('XBlock',dbl_ovrd);
      | iPos = get_param(gcb,'Position');
      | iWidth=iPos(3)-iPos(1); iHeight=iPos(4)-iPos(2);
      | iCx=iWidth/2;
      | iCy=iHeight/2;
      | [logoX, logoY] = xlogo(iPos);
      | [memX,memY] = memplot(iPos,min(depth,floor(iWidth/4)));
      | 
      | dataBPNum = 1;
      | dataBStr = '';
      | weBPNum = 1;
      | weBStr = '';
      | rstAPNum = 1;
      | rstAStr = '';
      | rstBPNum = 1;
      | rstBStr = '';
      | if(distributed_mem==0)
      |    dataBPNum = 5;
      |    dataBStr = 'data_B';
      |    weBPNum = 6;
      |    weBStr = 'we_B';
      |    if (latency==1)
      | 	   if (rst_a)
      | 		   rstAPNum = 7;
      | 		   rstAStr = 'rst_A';
      | 		   if (rst_b)
      | 	   			rstBPNum = 8;
      | 				rstBStr = 'rst_B';
      | 			end
      | 		else
      | 			if (rst_b)
      | 	   			rstBPNum = 7;
      | 				rstBStr = 'rst_B';
      | 			end
      | 		end
      |    end
      | end
      | 
      | voutAPNum = 1;
      | voutAStr = '';
      | voutBPNum = 1;
      | voutBStr = '';
      | doutBPNum=2;
      | if((mem_collision==1) && (distributed_mem==0) )
      |    voutAPNum = 2;
      |    voutAStr = 'vout_A';
      |    doutBPNum=3;
      |    voutBPNum = 4;
      |    voutBStr = 'vout_B';
      | end
      | 
      | % one time added for param list
      | useCore = 1;
      | dblOvrd = dbl_ovrd;
      | precision0 = 1;
      | precision1 = 1;
      | precision2 = 1;
      | precision3 = 1;
      | depthA = depth;
      | init = initVector;
      | write_mode_a = write_mode_A;
      | write_mode_b = write_mode_B;
      | initZero = init_zero;
      | explicitClk = explicit_period;
      | gen_core = 1;
      | 
      | % just pass everything to s-function
      | sfcn_mwsv__ = get_param(gcb, 'MaskWSVariables');
      | 
      | nport = get_param(gcbh, 'ports');
      | nin = nport(1);
      | nout = nport(2);
      mask Help: eval('xlWeb(xlhtmldoclink(''Dual Port RAM''))');
      mask StyleString: edit,edit,popup(Read After Write|Read Before Write|No Read On Write),popup(Read After Write|Read Before Write|No Read On Write),edit,checkbox,checkbox,checkbox,edit,checkbox,checkbox,edit,checkbox,edit,checkbox,checkbox,checkbox,checkbox,edit,checkbox
      mask Display:
      | patch([0 iWidth iWidth 0],[0 0 iHeight iHeight] ,bg);
      | patch([0 iWidth iWidth 0],[iCy-2 iCy-2 iCy+2 iCy+2] , .9* bg);
      | patch(logoX,logoY , fg);
      | port_label('input',1,'addr_A');
      | port_label('input',2,'data_A');
      | port_label('input',3,'we_A');
      | port_label('input',4,'addr_B');
      | port_label('input',dataBPNum,dataBStr);
      | port_label('input',weBPNum,weBStr);
      | port_label('input',rstAPNum,rstAStr);
      | port_label('input',rstBPNum,rstBStr);
      | port_label('output',1,'A');
      | port_label('output',doutBPNum,'B');
      | port_label('output',voutAPNum,voutAStr);
      | port_label('output',voutBPNum,voutBStr);
      | ;plot([0 0 iWidth iWidth 0], [0 iHeight iHeight 0 0]);
  Expression : S-Function  FunctionName=xldeprecated  Parameters=nin,nout  mask(Xilinx Expression Block){expression=a & b, precision=Full, arith_type=Unsigned, n_bits=8, bin_pt=2, align_bp=on, latency=0, explicit_period=off, period=1, en=off, dbl_ovrd=off, show_param=off, xl_area=[0, 0, 0, 0, 0, 0, 0], xl_use_area=off}
      mask prompts: arith_type "Output Type"; n_bits "Number of Bits"; bin_pt "Binary Point"; align_bp "Align Binary Point"; explicit_period "Use Explicit Sample Period"; period "Sample Period  (use -1 to inherit first known input period)"; en "Provide Enable Port"; dbl_ovrd "Override with Doubles"; show_param "---------------------- Show Implementation Parameters -----------------------------------------------------------------------------------"; xl_area "FPGA Area [Slices, FFs, BRAMs, LUTs, IOBs, Emb. Mults, TBUFs]"; xl_use_area "Use Area Above For Estimation"
      mask help:
      | BLOCK IS OUT OF DATE.
      |
      | This block is from an outdated copy of the Xilinx Blockset. Please run xlUpdateModel('<model-name>') to update to the latest version.
      mask init:
      | %remove these!
      | use_rpm = 0;
      | use_core = 0;
      | 
      | [port_names, vhdl_expr] = xlLogicalIdentifiers(expression);
      | num_inputs = length(port_names);
      | 
      | dprt = [1:num_inputs 1+zeros(1,33-num_inputs)];
      | dstr1='';dstr2='';dstr3='';dstr4='';dstr5='';dstr6='';dstr7='';dstr8='';dstr9='';dstr10='';
      | dstr11='';dstr12='';dstr12='';dstr13='';dstr14='';dstr15='';dstr16='';dstr17='';dstr18='';dstr19='';dstr20='';dstr21='';dstr22='';dstr23='';dstr24='';dstr25='';dstr26='';dstr27='';dstr28='';dstr29='';dstr30='';dstr31='';dstr32='';
      | 
      | if (num_inputs > 0) dstr1 = port_names{1}; end
      | if (num_inputs > 1) dstr2 = port_names{2}; end
      | if (num_inputs > 2) dstr3 = port_names{3}; end
      | if (num_inputs > 3) dstr4 = port_names{4}; end
      | if (num_inputs > 4) dstr5 = port_names{5}; end
      | if (num_inputs > 5) dstr6 = port_names{6}; end
      | if (num_inputs > 6) dstr7 = port_names{7}; end
      | if (num_inputs > 7) dstr8 = port_names{8}; end
      | if (num_inputs > 8) dstr9 = port_names{9}; end
      | if (num_inputs > 9) dstr10 = port_names{10}; end
      | if (num_inputs > 10) dstr11 = port_names{11}; end
      | if (num_inputs > 11) dstr12 = port_names{12}; end
      | if (num_inputs > 12) dstr13 = port_names{13}; end
      | if (num_inputs > 13) dstr14 = port_names{14}; end
      | if (num_inputs > 14) dstr15 = port_names{15}; end
      | if (num_inputs > 15) dstr16 = port_names{16}; end
      | if (num_inputs > 16) dstr17 = port_names{17}; end
      | if (num_inputs > 17) dstr18 = port_names{18}; end
      | if (num_inputs > 18) dstr19 = port_names{19}; end
      | if (num_inputs > 19) dstr20 = port_names{20}; end
      | if (num_inputs > 20) dstr21 = port_names{21}; end
      | if (num_inputs > 21) dstr22 = port_names{22}; end
      | if (num_inputs > 22) dstr23 = port_names{23}; end
      | if (num_inputs > 23) dstr24 = port_names{24}; end
      | if (num_inputs > 24) dstr25 = port_names{25}; end
      | if (num_inputs > 25) dstr26 = port_names{26}; end
      | if (num_inputs > 26) dstr27 = port_names{27}; end
      | if (num_inputs > 27) dstr28 = port_names{28}; end
      | if (num_inputs > 28) dstr29 = port_names{29}; end
      | if (num_inputs > 29) dstr30 = port_names{30}; end
      | if (num_inputs > 30) dstr31 = port_names{31}; end
      | if (num_inputs > 31) dstr32 = port_names{32}; end
      | 
      | [enPortNum,enPortStr] = xlport_en_rst(en,0,num_inputs+1);
      | 
      | [designRoot, family, part, speed, package, simulinkPeriod, sysclkPeriod, dbl_ovrd, trimVbit] = xlSysgenSettings(gcb,1,1);
      | operators = [' and'; 'nand'; '  or'; ' nor'; ' xor'; 'xnor'];
      | ostr = 'expr';
      | [bg,fg] = xlcmap_r3('XBlock',dbl_ovrd);
      | iPos = get_param(gcb,'Position');
      | iWidth=iPos(3)-iPos(1); iHeight=iPos(4)-iPos(2);
      | iCx=iWidth/2;
      | iCy=iHeight/2;
      | [logoX, logoY] = xlogo(iPos);
      | zstr=''; zpstr='';
      | if latency > 0
      |   zstr = 'z';
      |   zpstr = sprintf('-%d', latency);
      | end
      | zstrx = 0.45*iWidth-3; if (zstrx<3) zstrx=3; end
      | zstry = 0.36*iHeight-7; if (zstry<3) zstry=3; end
      | 
      | % one time added for param list
      | dblOvrd = dbl_ovrd;
      | numInputs = num_inputs;
      | useCore = use_core;
      | precision0 = precision;
      | z0 = [n_bits bin_pt arith_type 1 1 ];
      | explicitClk = explicit_period;
      | 
      | rpm = use_rpm;
      | hasEN = en;
      | 
      | % just pass everything to s-function
      | sfcn_mwsv__ = get_param(gcb, 'MaskWSVariables');
      | 
      | nport = get_param(gcbh, 'ports');
      | nin = nport(1);
      | nout = nport(2);
      mask Help: eval('xlWeb(xlhtmldoclink(''Expression''))');
      mask StyleString: edit,popup(Full|User Defined),popup(Unsigned|Signed  (2's comp)),edit,edit,checkbox,edit,checkbox,edit,checkbox,checkbox,checkbox,edit,checkbox
      mask Display:
      | patch([0 iWidth iWidth 0],[0 0 iHeight iHeight] ,bg);
      | patch(logoX,logoY,  fg);
      | disp(expression);
      | text(zstrx,zstry,zstr);
      | text(zstrx+5,zstry+5,zpstr);
      | 
      | 
      | ;plot([0 0 iWidth iWidth 0], [0 iHeight iHeight 0 0]);
      | 
      | port_label('input',dprt(1), dstr1);
      | port_label('input',dprt(2), dstr2);
      | port_label('input',dprt(3), dstr3);
      | port_label('input',dprt(4), dstr4);
      | port_label('input',dprt(5), dstr5);
      | port_label('input',dprt(6), dstr6);
      | port_label('input',dprt(7), dstr7);
      | port_label('input',dprt(8), dstr8);
      | port_label('input',dprt(9), dstr9);
      | port_label('input',dprt(10), dstr10);
      | port_label('input',dprt(11), dstr11);
      | port_label('input',dprt(12), dstr12);
      | port_label('input',dprt(13), dstr13);
      | port_label('input',dprt(14), dstr14);
      | port_label('input',dprt(15), dstr15);
      | port_label('input',dprt(16), dstr16);
      | port_label('input',dprt(17), dstr17);
      | port_label('input',dprt(18), dstr18);
      | port_label('input',dprt(19), dstr19);
      | port_label('input',dprt(20), dstr20);
      | port_label('input',dprt(21), dstr21);
      | port_label('input',dprt(22), dstr22);
      | port_label('input',dprt(23), dstr23);
      | port_label('input',dprt(24), dstr24);
      | port_label('input',dprt(25), dstr25);
      | port_label('input',dprt(26), dstr26);
      | port_label('input',dprt(27), dstr27);
      | port_label('input',dprt(28), dstr28);
      | port_label('input',dprt(29), dstr29);
      | port_label('input',dprt(30), dstr30);
      | port_label('input',dprt(31), dstr31);
      | port_label('input',dprt(32), dstr32);
      | 
      | port_label('input',enPortNum,enPortStr);
  FDATool : Subsystem  mask(Xilinx FDATool Interface){}
      mask help: Digital filter design using FDATool GUI.
      mask init:
      | [bg,fg] = xlcmap_r3('XTool');
      | iPos = get_param(gcb,'Position');
      | iWidth=iPos(3)-iPos(1); iHeight=iPos(4)-iPos(2);
      | iCx=iWidth/2;
      | iCy=iHeight/2;
      | [logoX, logoY] = xlogo(iPos);
      | 
      | try
      | 	foo = dspblkfdatool('getIcon',gcb);
      | 	foo = foo(1:ceil(length(foo)/512):end);
      | catch
      | 	foo = [ 0.7500 0.7489 0.7464 0.7446 0.7452 0.7477 0.7497 0.7496 0.7474 0.7450 0.7448 0.7471 0.7495 0.7498 0.7476 0.7451 0.7448 0.7471 0.7496 0.7497 0.7474 0.7449 0.7450 0.7477 0.7499 0.7483 0.7407 0.7257 0.7020 0.6676 0.6184 0.5443 0.3680 0.3372 0.3077 0.3674 0.3287 0.3629 0.3389 0.3631 0.3301 0.3659 0.2983 0.3681 0.2801 0.3661 0.3361 0.3575 0.3575 0.3350 0.3667 0.2177 0.3672 0.3317 0.3579 0.3582 0.3307 0.3675 0.2581 0.3659 0.3420 0.3524 0.3627 0.3096];
      |   end
      | 
      | foox = 5+.9*iWidth * (1:length(foo))/length(foo); 
      | foo = 5+.9*foo * iHeight;
      settings: OpenFcn=modelName = get_param(bdroot, 'name');h = errordlg(sprintf(['This block is from an outdated copy of the Xilinx Blockset.\nPlease run xlUpdateModel(''' modelName ''') to update this design.']), 'Update Required');
      mask Help: eval('xlWeb(xlhtmldoclink(''FDATool''))');
      mask Display:
      | patch([0 iWidth iWidth 0],[0 0 iHeight iHeight] , bg);
      | patch(logoX,logoY, fg);
      | 
      | plot([0 0 iWidth iWidth 0], [0 iHeight iHeight 0 0]);
      | plot(foox,foo);
      | text(5, iHeight-8,'FDATool');
  FFT : S-Function  FunctionName=xldeprecated  Parameters=nin,nout  mask(Xilinx Fast Fourier Transform){n=64, mem=Triple, scale_mode=1/N, oflw_inv=on, explicit_period=off, period=1, rst=off, dbl_ovrd=off, show_param=off, gen_core=off, xl_area=[0, 0, 0, 0, 0, 0, 0], xl_use_area=off}
      mask prompts: n "Number of Sample Points (N)"; mem "Memory Usage"; scale_mode "Scale Output By"; oflw_inv "Invalidate Transform on Overflow"; explicit_period "Use Explicit Sample Period"; period "Sample Period  (use -1 to inherit first known input period)"; rst "Provide Reset Port"; dbl_ovrd "Override with Doubles"; show_param "---------------------- Show Implementation Parameters -----------------------------------------------------------------------------------"; gen_core "Generate Core"; xl_area "FPGA Area [Slices, FFs, BRAMs, LUTs, IOBs, Emb. Mults, TBUFs]"; xl_use_area "Use Area Above For Estimation"
      mask help:
      | BLOCK IS OUT OF DATE.
      |
      | This block is from an outdated copy of the Xilinx Blockset. Please run xlUpdateModel('<model-name>') to update to the latest version.
      mask init:
      | npts = sscanf(n,'%f');
      | [designRoot, family, part, speed, package, simulinkPeriod, sysclkPeriod, dbl_ovrd, trimVbit] = xlSysgenSettings(gcb,1,0);
      | trimVbit=1;
      | [bg,fg] = xlcmap_r3('XBlock',dbl_ovrd);
      |  [enPortNum,enPortStr,rstPortNum,rstPortStr,portDir] = xlport_en_rst(0,rst,5);
      | 
      | iPos = get_param(gcb,'Position');
      | iWidth=iPos(3)-iPos(1); iHeight=iPos(4)-iPos(2);
      | iCx=iWidth/2;
      | iCy=iHeight/2;
      | [logoX, logoY] = xlogo(iPos);
      | 
      | 
      | 
      | % one time added for param list
      | precision0 = 1;
      | precision1 = 1;
      | precision2 = 1;
      | precision3 = 1;
      | precision4 = 1;
      | latency = 1;
      | memory_usage = mem;
      | explicitClk = explicit_period;
      | useCore = 1;
      | hasRST = rst;
      | dblOvrd = dbl_ovrd;
      | gen_core = 1;
      | % just pass everything to s-function
      | sfcn_mwsv__ = get_param(gcb, 'MaskWSVariables');
      | 
      | nport = get_param(gcbh, 'ports');
      | nin = nport(1);
      | nout = nport(2);
      mask Help: eval('xlWeb(xlhtmldoclink(''FFT''))');
      mask StyleString: popup(16|64|256|1024),popup(Single|Double|Triple),popup(1/N|1/(2N)),checkbox,checkbox,edit,checkbox,checkbox,checkbox,checkbox,edit,checkbox
      mask Display:
      | patch([0 iWidth iWidth 0],[0 0 iHeight iHeight] , bg);
      | patch(logoX,logoY , fg);
      | port_label(portDir,rstPortNum,rstPortStr);
      | port_label('input',1,'xn_r');
      | port_label('input',2,'xn_i');
      | port_label('input',3,'vin');
      | port_label('input',4,'inv');
      | port_label('output',1,'Xk_r');
      | port_label('output',2,'Xk_i');
      | port_label('output',3,'vout');
      | port_label('output',4,'done');
      | port_label('output',5,'rfd');
      | ;plot([0 0 iWidth iWidth 0], [0 iHeight iHeight 0 0]);
  FFTx : S-Function  FunctionName=xldeprecated  Parameters=nin,nout  mask(Xilinx Fast Fourier Transform){arch=Pipelined Streaming I/O, npts=512, scaling=Unscaled, rounding=Truncation, tf_width=8, op_order=Bit Reversed Order, twiddle_mem_type=Block RAM, data_mem_type=Block RAM, num_bram_stages=3, explicit_period=off, period=-1, use_dsp48=off, en_n=off, has_ovflo=off, rst=off, en=off, dbl_ovrd=off, show_param=off, gen_core=off, xl_area=[0, 0, 0, 0, 0, 0, 0], xl_use_area=off}
      mask prompts: arch "Implementation"; npts "Number of Sample Points (N)"; rounding "Rounding Mode"; tf_width "Phase Factor Bit Width"; op_order "Output Ordering"; twiddle_mem_type "Phase Factor Memory Type"; data_mem_type "Data Memory Type"; num_bram_stages "Number of Stages Using Block RAM"; explicit_period "Use Explicit Sample Period"; period "Sample Period  (use -1 to inherit first known input period)"; use_dsp48 "Optimize for Speed Using DSP48"; en_n "Enable Dynamic Transform Size"; has_ovflo "Provide Overflow Port"; rst "Provide Reset Port"; en "Provide Enable Port"; dbl_ovrd "Override with Doubles"; show_param "---------------------- Show Implementation Parameters -----------------------------------------------------------------------------------"; gen_core "Generate Core"; xl_area "FPGA Area [Slices, FFs, BRAMs, LUTs, IOBs, Emb. Mults, TBUFs]"; xl_use_area "Use Area Above For Estimation"
      mask help:
      | BLOCK IS OUT OF DATE.
      |
      | This block is from an outdated copy of the Xilinx Blockset. Please run xlUpdateModel('<model-name>') to update to the latest version.
      mask init:
      | xlmeta;
      | [designRoot, family, part, speed, package, simulinkPeriod, sysclkPeriod, dbl_ovrd, trimVbit] = xlSysgenSettings(gcb,1,0);
      | xlISEVer = xlGetISEVer;
      | c_family = 0;
      | if(strcmp(family,'Virtex4'))
      | 	c_family = 1;
      | end
      | [bg,fg] = xlcmap_r3('XBlock',dbl_ovrd);
      | iPos = get_param(gcb,'Position');
      | iWidth=iPos(3)-iPos(1); iHeight=iPos(4)-iPos(2);
      | iCx=iWidth/2;
      | iCy=iHeight/2;
      | [logoX, logoY] = xlogo(iPos);
      | 
      | % one time added for param list
      | numinputs = 5;
      | unloadNum = 1;
      | unloadStr = '';
      | if ((arch > 1) & (arch < 4))
      | 	numinputs = numinputs+1;
      | 	unloadNum = numinputs;
      | 	unloadStr = 'unload';
      | end
      | scaleschNum = 1;
      | scaleschStr = '';
      | scalesch_weNum = 1;
      | scalesch_weStr = '';
      | if (scaling == 2)
      | 	numinputs = numinputs+1;
      | 	scaleschNum = numinputs;
      | 	scaleschStr = 'scale_sch';
      | 	numinputs = numinputs+1;
      | 	scalesch_weNum = numinputs;
      | 	scalesch_weStr = 'scale_sch_we';
      | end
      | NNum = 1;
      | NStr = '';
      | N_WENum = 1;
      | N_WEStr = '';
      | if (en_n == 1)
      | 	numinputs = numinputs+1;
      | 	NNum = numinputs;
      | 	NStr = 'nfft';
      | 	numinputs = numinputs+1;
      | 	N_WENum = numinputs;
      | 	N_WEStr = 'nfft_we';
      | end
      | numinputs = numinputs+1;
      |  [enPortNum,enPortStr,rstPortNum,rstPortStr,portDir] = xlport_en_rst(en,rst,numinputs);
      | 
      | % Number of outputs start with 9
      | numoutputs = 9;
      | expNum = 1;
      | expStr = '';
      | if (scaling == 3)
      | 	numoutputs = numoutputs+1;
      | 	expNum = numoutputs;
      | 	expStr = 'blk_exp';
      | end
      | ovfloNum = 1;
      | ovfloStr = '';
      | if (scaling ==2)
      | 	if ((arch == 1) | (has_ovflo == 1))
      | 		numoutputs = numoutputs+1;
      | 		ovfloNum = numoutputs;
      | 		ovfloStr = 'ovflo';
      | 	end
      | end
      | numoutputs = numoutputs+1;
      | rfdNum = numoutputs;
      | numoutputs = numoutputs+1;
      | busyNum = numoutputs;
      | 
      | % one time added for param list
      | precision0 = 1;
      | precision1 = 1;
      | precision2 = 1;
      | precision3 = 1;
      | precision4 = 1;
      | precision5 = 1;
      | precision6 = 1;
      | precision7 = 1;
      | precision8 = 1;
      | precision9 = 1;
      | 
      | iPos = get_param(gcb,'Position');
      | iWidth=iPos(3)-iPos(1); iHeight=iPos(4)-iPos(2);
      | iCx=iWidth/2;
      | iCy=iHeight/2;
      | [logoX, logoY] = xlogo(iPos);
      | 
      | latency = 1;
      | explicitClk = explicit_period;
      | useCore = 1;
      | hasRST = rst;
      | hasEN = en;
      | dblOvrd = dbl_ovrd;
      | 
      | xlv2fft_dll=[ xlFindSysgenRoot '\bin\xlv2fft_v3_1.dll'];
      | 
      | % just pass everything to s-function
      | sfcn_mwsv__ = get_param(gcb, 'MaskWSVariables');
      | %Warning For Radix-4 Streaming I/O
      | if (arch ==1)
      | 	disp('Warning: Radix-4 Streaming I/O will be obsoleted');
      | 	disp('         in subsequent release of FFTx block.');
      | 	disp('         Use the Pipelined Streaming I/O option');
      | 	disp('         for implementing FFT in streaming mode.');
      | end
      | nport = get_param(gcbh, 'ports');
      | nin = nport(1);
      | nout = nport(2);
      mask Help: eval('xlWeb(xlhtmldoclink(''FFTx''))');
      mask StyleString: popup(Radix-4 Streaming I/O|Radix-4 Burst I/O|Radix-2 Minimum Resources|Pipelined Streaming I/O),popup(8|16|32|64|128|256|512|1024|2048|4096|8192|16384|32768|65536),popup(Unscaled|Scaled|Block Floating Point),popup(Truncation|Convergent Rounding),popup(8|12|16|20|24),popup(Bit Reversed Order|Natural Order),popup(Block RAM|Distributed RAM),popup(Block RAM|Distributed RAM),popup(0|1|2|3|4|5|6|7|8|9|10|11|12|13),checkbox,edit,checkbox,checkbox,checkbox,checkbox,checkbox,checkbox,checkbox,checkbox,edit,checkbox
      mask Display:
      | patch([0 iWidth iWidth 0],[0 0 iHeight iHeight] , bg);
      | patch(logoX,logoY , fg);
      | port_label(portDir,rstPortNum,rstPortStr);
      | port_label('input',1,'xn_re');
      | port_label('input',2,'xn_im');
      | port_label('input',3,'start');
      | port_label('input',4,'fwd');
      | port_label('input',5,'fwd_we');
      | port_label('input',unloadNum,unloadStr);
      | port_label('input',scaleschNum,scaleschStr);
      | port_label('input',scalesch_weNum,scalesch_weStr);
      | port_label('input',NNum,NStr);
      | port_label('input',N_WENum,N_WEStr);
      | port_label(portDir,rstPortNum,rstPortStr);
      | port_label(portDir,enPortNum,enPortStr);
      | port_label('output',1,'xk_re');
      | port_label('output',2,'xk_im');
      | port_label('output',3,'xn_index');
      | port_label('output',4,'xk_index');
      | port_label('output',5,'rfd');
      | port_label('output',6,'busy');
      | port_label('output',7,'vout');
      | port_label('output',8,'edone');
      | port_label('output',9,'done');
      | port_label('output',expNum,expStr);
      | port_label('output',ovfloNum,ovfloStr);
      | ;plot([0 0 iWidth iWidth 0], [0 iHeight iHeight 0 0]);
  FIFO : S-Function  FunctionName=xldeprecated  Parameters=nin,nout  mask(Xilinx Synchronous FIFO){depth=16, percent_nbits=1, store_only_valid=on, init_zero=on, explicit_period=off, period=1, rst=off, en=off, use_almost_empty=off, almost_empty_offset=6, use_almost_full=off, almost_full_offset=6, dbl_ovrd=off, show_param=off, mem_type=Block RAM, gen_core=off, xl_area=[0, 0, 0, 0, 0, 0, 0], xl_use_area=off}
      mask prompts: percent_nbits "Bits of Precision to Use for "Percent Full" Signal"; store_only_valid "Store Only Valid Data"; init_zero "Zero Initial Output  (otherwise NaN)"; explicit_period "Use Explicit Sample Period"; period "Sample Period  (use -1 to inherit first known input period)"; rst "Provide Reset Port"; en "Provide Enable Port"; use_almost_empty "Provide Almost Empty Port"; almost_empty_offset "Almost Empty Offset"; use_almost_full "Provide Almost Full Port"; almost_full_offset "Almost Full Offset"; dbl_ovrd "Override with Doubles"; show_param "---------------------- Show Implementation Parameters -----------------------------------------------------------------------------------"; mem_type "Memory Type"; gen_core "Generate Core"; xl_area "FPGA Area [Slices, FFs, BRAMs, LUTs, IOBs, Emb. Mults, TBUFs]"; xl_use_area "Use Area Above For Estimation"
      mask help:
      | BLOCK IS OUT OF DATE.
      |
      | This block is from an outdated copy of the Xilinx Blockset. Please run xlUpdateModel('<model-name>') to update to the latest version.
      mask init:
      | edepth = 2^(3+depth);
      | countWidth = percent_nbits;
      | if (mem_type ~= 3)
      | 	dmem = mem_type - 1;
      | 	useCore = 1;
      | 	gen_core = 1;
      | else
      | 	dmem = 0;
      | 	useCore = 0;
      | 	gen_core = 0;
      | end
      | [designRoot, family, part, speed, package, simulinkPeriod, sysclkPeriod, dbl_ovrd, trimVbit] = xlSysgenSettings(gcb,1,1);
      | [bg,fg] = xlcmap_r3('XBlock',dbl_ovrd);
      | iPos = get_param(gcb,'Position');
      | iWidth=iPos(3)-iPos(1); iHeight=iPos(4)-iPos(2);
      | iCx=iWidth/2;
      | iCy=iHeight/2;
      | [logoX, logoY] = xlogo(iPos);
      | [enPortNum,enPortStr,rstPortNum,rstPortStr] = xlport_en_rst(en,rst,4);
      | % one time added for param list
      | hasRST = rst;
      | hasEN = en;
      | hasALMOST_FULL = use_almost_full;
      | hasALMOST_EMPTY = use_almost_empty;
      | latency = 1;
      | dblOvrd = dbl_ovrd;
      | precision0 = 1;
      | precision1 = 1;
      | precision2 = 1;
      | precision3 = 1;
      | depth = edepth;
      | vOnly = store_only_valid;
      | initZero = init_zero;
      | distributed_mem = dmem;
      | explicitClk = explicit_period;
      | 
      | 
      | % Output Port Management
      | 
      | opt_ports = 3; % default starting port num for optional ports
      | 
      | % Initialize output port strings
      | percent_full_str = 'dout';
      | full_str = 'dout';
      | almost_empty_str = 'dout';
      | almost_full_str = 'dout';
      | 
      | % Initialize output port numbers
      | percent_full_num = 1;
      | full_num = 1;
      | almost_empty_num = 1;
      | almost_full_num = 1;
      | 
      | % Determine output ports
      | port_index = opt_ports;
      | 
      | if (mem_type ~= 3)
      | 	percent_full_num = port_index;
      | 	percent_full_str = '%full';
      | 	port_index = port_index + 1;
      | end
      | 
      | full_num = port_index;
      | full_str = 'full';
      | port_index = port_index + 1;
      | 
      | if (mem_type == 3)
      | 	if (use_almost_empty)
      | 		almost_empty_num = port_index;
      | 		almost_empty_str = 'almost_empty';
      | 		port_index = port_index + 1;
      | 	end
      | 	if (use_almost_full)
      | 		almost_full_num = port_index;
      | 		almost_full_str = 'almost_full';
      | 		port_index = port_index + 1;
      | 	end
      | end
      | 
      | 
      | % just pass everything to s-function
      | sfcn_mwsv__ = get_param(gcb, 'MaskWSVariables');
      | 
      | nport = get_param(gcbh, 'ports');
      | nin = nport(1);
      | nout = nport(2);
      mask Help: eval('xlWeb(xlhtmldoclink(''FIFO''))');
      mask StyleString: popup(16|32|64|128|256|512|1K|2K|4K|8K|16K|32K|64K),popup(1|2|3|4|5),checkbox,checkbox,checkbox,edit,checkbox,checkbox,checkbox,edit,checkbox,edit,checkbox,checkbox,popup(Block RAM|Distributed RAM|Embedded FIFO),checkbox,edit,checkbox
      mask Display:
      | patch([0 iWidth iWidth 0],[0 0 iHeight iHeight] , bg);
      | patch(logoX,logoY , fg);
      | 
      | port_label('input',1,'din');
      | port_label('input',2,'we');
      | port_label('input',3,'re');
      | port_label('input',enPortNum,enPortStr);
      | port_label('input',rstPortNum,rstPortStr);
      | port_label('output',1,'dout');
      | port_label('output',2,'empty');
      | port_label('output',percent_full_num,percent_full_str);
      | port_label('output',full_num,full_str);
      | port_label('output',almost_empty_num,almost_empty_str);
      | port_label('output',almost_full_num,almost_full_str);
      | 
      | ;plot([0 0 iWidth iWidth 0], [0 iHeight iHeight 0 0]);
  FIR : S-Function  FunctionName=xldeprecated  Parameters=nin,nout  mask(Xilinx Finite Impulse Response Filter){coef=[1 -1], structure=Inferred from Coefficients, coef_n_bits=8, coef_bin_pt=6, coef_arith_type=Signed  (2's complement), num_channels=1, serial_input=off, polyphase_behavior=Single Rate:  sample in - sample out, latency=1, over_sample=1, explicit_period=off, period=1, reload=off, valids=off, dbl_ovrd=off, show_param=off, gen_core=off, xl_area=[0, 0, 0, 0, 0, 0, 0], xl_use_area=off}
      mask prompts: coef "Coefficients"; structure "Coefficient Structure"; coef_n_bits "Number of Bits per Coefficient  (always treated as signed)"; coef_bin_pt "Binary Point for Coefficients"; coef_arith_type "Arithmetic Type for Coefficients"; num_channels "Number of Channels"; serial_input "Serial Input"; polyphase_behavior "Polyphase Behavior"; over_sample "Hardware Over-Sampling Rate"; explicit_period "Use Explicit Sample Period"; period "Sample Period"; reload "Provide Coefficient Reload Ports"; valids "Provide Valid Ports"; dbl_ovrd "Override with Doubles"; show_param "---------------------- Show Implementation Parameters -----------------------------------------------------------------------------------"; gen_core "Generate Core"; xl_area "FPGA Area [Slices, FFs, BRAMs, LUTs, IOBs, Emb. Mults, TBUFs]"; xl_use_area "Use Area Above For Estimation"
      mask help:
      | BLOCK IS OUT OF DATE.
      |
      | This block is from an outdated copy of the Xilinx Blockset. Please run xlUpdateModel('<model-name>') to update to the latest version.
      mask init:
      | if(~serial_input)
      |  dstr = sprintf('%d tap',length(coef));
      |  dstr2 = '';
      | else 
      |  dstr = sprintf('%d tap',length(coef));
      |  dstr2 = sprintf('%d channel',num_channels);
      | end
      | if(~serial_input)
      |  dprt = [1:num_channels 1+zeros(1,8-num_channels)];
      |  vprt = 1; if (valids) vprt = num_channels+1; end;
      |  lprt0 = 1; lprt1 =1; lprt2 = 1;
      |  rfdprt = 1;
      |  seli_port = 1;
      |  selo_port = 1;
      |  if (reload)
      |    lprt0 = num_channels+1;
      |    rfdprt = num_channels+1;
      |    if (valids) lprt0 = lprt0 + 1; rfdprt = rfdprt+1; end;
      |    lprt1 = lprt0 + 1; lprt2 = lprt1 + 1;
      |  end;
      | else
      |  dprt = [1:1 1+zeros(1,7)];
      |  vprt = 2; % there is a vin/vout port
      |  lprt0 = 1; lprt1 =1; lprt2 = 1; rfdprt = 3;
      |  seli_port = 4; selo_port = 5;
      |  if(reload)
      | 	 lprt0 = 3; lprt1 = 4; lprt2 = 5;
      |  end 
      | end
      | xstr0 = 'xn'; xstr1 = ''; xstr2 = ''; xstr3 = ''; xstr4 = ''; xstr5 = ''; xstr6 = ''; xstr7 = '';
      | ystr0 = 'yn'; ystr1 = ''; ystr2 = ''; ystr3 = ''; ystr4 = ''; ystr5 = ''; ystr6 = ''; ystr7 = '';
      | vinstr = ''; voutstr = '';
      | loadstr0 = ''; loadstr1 = ''; loadstr2 = '';
      | selistr = '';selostr = '';
      | rfdstr = '';
      | if(~serial_input)
      |   if (num_channels > 1) xstr0 = 'xn0'; xstr1 = 'xn1'; ystr0 = 'yn0'; ystr1 = 'yn1'; end;
      |   if (num_channels > 2) xstr2 = 'xn2'; ystr2 = 'yn2'; end;
      |   if (num_channels > 3) xstr3 = 'xn3'; ystr3 = 'yn3'; end;
      |   if (num_channels > 4) xstr4 = 'xn4'; ystr4 = 'yn4'; end;
      |   if (num_channels > 5) xstr5 = 'xn5'; ystr5 = 'yn5'; end;
      |   if (num_channels > 6) xstr6 = 'xn6'; ystr6 = 'yn6'; end;
      |   if (num_channels > 7) xstr7 = 'xn7'; ystr7 = 'yn7'; end;
      |   if (valids) vinstr = 'vin'; voutstr = 'vout'; end;
      |   if (reload) loadstr0 = 'coef'; loadstr1 = 'load'; loadstr2 = 'coef_we';
      |                rfdstr = 'rfd'; end;
      | else
      |   xstr0 = 'x'; ystr0 = 'y';
      |   vinstr = 'vin'; voutstr = 'vout'; rfdstr = 'rfd';
      |   selistr = 'sel_in'; selostr = 'sel_out';
      |   if (reload) loadstr0 = 'coef'; loadstr1 = 'load'; loadstr2 = 'coef_we';
      |                rfdstr = 'rfd'; end;
      | end
      | polyphase = polyphase_behavior - 7;
      | [designRoot, family, part, speed, package, simulinkPeriod, sysclkPeriod, dbl_ovrd, trimVbit] = xlSysgenSettings(gcb,1,0);
      | trimVbit=1;
      | [bg,fg] = xlcmap_r3('XBlock',dbl_ovrd);
      | iPos = get_param(gcb,'Position');
      | iWidth=iPos(3)-iPos(1); iHeight=iPos(4)-iPos(2);
      | iCx=iWidth/2;
      | iCy=iHeight/2;
      | [logoX, logoY] = xlogo(iPos);
      | 
      | % one time added for param list
      | dblOvrd = dbl_ovrd;
      | useCore = 1;
      | precision0 = 1;
      | precision1 = 1;
      | precision2 = 1;
      | precision3 = 1;
      | precision4 = 1;
      | precision5 = 1;
      | precision6 = 1;
      | precision7 = 1;
      | precision8 = 1;
      | precision9 = 1;
      | hasValids = valids;
      | %force the usage of valids if not internal muxing
      | if(serial_input) hasValids = 1; end;
      | coefProto = [coef_n_bits coef_bin_pt 2 2 2];
      | numChan = num_channels;
      | overSample = over_sample;
      | explicitClk = explicit_period;
      | gen_core = 1;
      | if(serial_input == 1)
      | 	internal_mux = 0;
      | else
      | 	internal_mux = 1;
      | end
      | % just pass everything to s-function
      | sfcn_mwsv__ = get_param(gcb, 'MaskWSVariables');
      | 
      | nport = get_param(gcbh, 'ports');
      | nin = nport(1);
      | nout = nport(2);
      mask Help: eval('xlWeb(xlhtmldoclink(''FIR''))');
      mask StyleString: edit,popup(Inferred from Coefficients|None|Symmetric|Negative Symmetric|Half-Band Filter|Interpolated FIR),edit,edit,popup(Unsigned|Signed  (2's complement)),popup(1|2|3|4|5|6|7|8),checkbox,popup(Decimate:  8:1 (samples in:out)|Decimate:  7:1 (samples in:out)|Decimate:  6:1 (samples in:out)|Decimate:  5:1 (samples in:out)|Decimate:  4:1 (samples in:out)|Decimate:  3:1 (samples in:out)|Decimate:  2:1 (samples in:out)|Single Rate:  sample in - sample out|Interpolate:  1:2 (samples in:out)|Interpolate:  1:3 (samples in:out)|Interpolate:  1:4 (samples in:out)|Interpolate:  1:5 (samples in:out)|Interpolate:  1:6 (samples in:out)|Interpolate:  1:7 (samples in:out)|Interpolate:  1:8 (samples in:out)),edit,edit,checkbox,edit,checkbox,checkbox,checkbox,checkbox,checkbox,edit,checkbox
      mask Display:
      | patch([0 iWidth iWidth 0],[0 0 iHeight iHeight] , bg);
      | patch(logoX,logoY , fg);
      | text(iCx/1.4,iCy+2,dstr);
      | text((iCx/1.4)-10,iCy-10,dstr2);
      | 
      | plot([0 0 iWidth iWidth 0], [0 iHeight iHeight 0 0]);
      | 
      | port_label('input',dprt(1), xstr0);
      | port_label('input',dprt(2), xstr1);
      | port_label('input',dprt(3), xstr2);
      | port_label('input',dprt(4), xstr3);
      | port_label('input',dprt(5), xstr4);
      | port_label('input',dprt(6), xstr5);
      | port_label('input',dprt(7), xstr6);
      | port_label('input',dprt(8), xstr7);
      | port_label('output',dprt(1),ystr0);
      | port_label('output',dprt(2),ystr1);
      | port_label('output',dprt(3),ystr2);
      | port_label('output',dprt(4),ystr3);
      | port_label('output',dprt(5),ystr4);
      | port_label('output',dprt(6),ystr5);
      | port_label('output',dprt(7),ystr6);
      | port_label('output',dprt(8),ystr7);
      | port_label('input',vprt,vinstr);
      | port_label('output',vprt,voutstr);
      | port_label('input',lprt0,loadstr0);
      | port_label('input',lprt1,loadstr1);
      | port_label('input',lprt2,loadstr2);
      | port_label('output',rfdprt, rfdstr);
      | port_label('output',seli_port, selistr);
      | port_label('output',selo_port, selostr);
  From FIFO : S-Function  FunctionName=xldeprecated  Parameters=nin,nout  mask(Xilinx Shared Memory Based From FIFO){shared_memory_name='Bar', arith_type=Unsigned, n_bits=8, bin_pt=0, percent_nbits=1, explicit_period=off, period=1, dbl_ovrd=off, show_param=off, mem_type=Block RAM, xl_area=[0, 0, 0, 0, 0, 0, 0], xl_use_area=off, core_version=1.1}
      mask prompts: shared_memory_name "Shared Memory Name"; arith_type "Arithmetic Type"; n_bits "Number of Bits"; bin_pt "Binary Point Position"; percent_nbits "Bits of Precision to Use for "Percent Full" Signal"; explicit_period "Use Explicit Sample Period"; period "Sample Period  (use -1 to inherit first known input period)"; dbl_ovrd "Override with Doubles"; show_param "---------------------- Show Implementation Parameters -----------------------------------------------------------------------------------"; mem_type "Memory Type"; xl_area "FPGA Area [Slices, FFs, BRAMs, LUTs, IOBs, Emb. Mults, TBUFs]"; xl_use_area "Use Area Above For Estimation"; core_version "Core Version"
      mask help:
      | BLOCK IS OUT OF DATE.
      |
      | This block is from an outdated copy of the Xilinx Blockset. Please run xlUpdateModel('<model-name>') to update to the latest version.
      mask init:
      | dmem = mem_type - 1;
      | [designRoot, family, part, speed, package, simulinkPeriod, sysclkPeriod, dbl_ovrd, trimVbit] = xlSysgenSettings(gcb,1,1);
      | [bg,fg] = xlcmap_r3('Shmem',dbl_ovrd);
      | iPos = get_param(gcb,'Position');
      | iWidth=iPos(3)-iPos(1); iHeight=iPos(4)-iPos(2);
      | iCx=iWidth/2;
      | iCy=iHeight/2;
      | [logoX, logoY] = xlogo(iPos);
      | % one time added for param list
      | countWidth = sscanf(percent_nbits,'%f');
      | latency = 1;
      | dblOvrd = dbl_ovrd;
      | useCore = 1;
      | precision0 = 2;
      | precision1 = 2;
      | z0 = [n_bits bin_pt arith_type  1 1];
      | z1 = [countWidth countWidth 1 1 1];
      | explicitClk = explicit_period;
      | 
      | % just pass everything to s-function
      | sfcn_mwsv__ = get_param(gcb, 'MaskWSVariables');
      | 
      | nport = get_param(gcbh, 'ports');
      | nin = nport(1);
      | nout = nport(2);
      settings: AttributesFormatString=<< %<shared_memory_name> >>
      mask Help: eval('xlWeb(xlhtmldoclink(''From FIFO''))');
      mask StyleString: edit,popup(Unsigned|Signed  (2's comp)),edit,edit,popup(1|2|3|4|5|6|7|8|9|10),checkbox,edit,checkbox,checkbox,popup(Block RAM|Distributed RAM|FIFO16),edit,checkbox,edit
      mask Display:
      | patch([0 iWidth iWidth 0],[0 0 iHeight iHeight] , bg);
      | patch(logoX,logoY , fg);
      | port_label('input',1,'re');
      | port_label('output',1,'dout');
      | port_label('output',2,'%full');
      | port_label('output',3,'empty');
      | 
      | plot([0 0 iWidth iWidth 0], [0 iHeight iHeight 0 0]);
  From Register : S-Function  FunctionName=xldeprecated  Parameters=nin,nout  mask(Xilinx Shared Memory based From Register){shared_memory_name='Bar', arith_type=Unsigned, n_bits=8, bin_pt=0, explicit_period=off, period=1, dbl_ovrd=off, show_param=off, xl_area=[0, 0, 0, 0, 0, 0, 0], xl_use_area=off}
      mask prompts: shared_memory_name "Shared Memory Name"; arith_type "Arithmetic Type"; n_bits "Number of Bits"; bin_pt "Binary Point Position"; explicit_period "Use Explicit Sample Period"; period "Sample Period"; dbl_ovrd "Override with Doubles"; show_param "---------------------- Show Implementation Parameters -----------------------------------------------------------------------------------"; xl_area "FPGA Area [Slices, FFs, BRAMs, LUTs, IOBs, Emb. Mults, TBUFs]"; xl_use_area "Use Area Above For Estimation"
      mask help:
      | BLOCK IS OUT OF DATE.
      |
      | This block is from an outdated copy of the Xilinx Blockset. Please run xlUpdateModel('<model-name>') to update to the latest version.
      mask init:
      | [designRoot, family, part, speed, package, simulinkPeriod, sysclkPeriod, dbl_ovrd, trimVbit] = xlSysgenSettings(gcb,1,1);
      | [bg,fg] = xlcmap_r3('Shmem',dbl_ovrd);
      | iPos = get_param(gcb,'Position');
      | iWidth=iPos(3)-iPos(1); iHeight=iPos(4)-iPos(2);
      | iCx=iWidth/2;
      | iCy=iHeight/2;
      | [logoX, logoY] = xlogo(iPos);
      | % one time added for param list
      | latency = 0;
      | dblOvrd = dbl_ovrd;
      | precision0 = 2;
      | z0 = [n_bits bin_pt arith_type  1 1];
      | explicitClk = explicit_period;
      | 
      | % just pass everything to s-function
      | sfcn_mwsv__ = get_param(gcb, 'MaskWSVariables');
      | 
      | nport = get_param(gcbh, 'ports');
      | nin = nport(1);
      | nout = nport(2);
      settings: AttributesFormatString=<< %<shared_memory_name> >>
      mask Help: eval('xlWeb(xlhtmldoclink(''From Register''))');
      mask StyleString: edit,popup(Unsigned|Signed  (2's comp)),edit,edit,checkbox,edit,checkbox,checkbox,edit,checkbox
      mask Display:
      | patch([0 iWidth iWidth 0],[0 0 iHeight iHeight] , bg);
      | patch(logoX,logoY , fg);
      | 
      | port_label('output',1,'dout');
      | 
      | plot([0 0 iWidth iWidth 0], [0 iHeight iHeight 0 0]);
  Gateway In : S-Function  FunctionName=xldeprecated  Parameters=nin,nout  mask(Xilinx Gateway In){arith_type=Signed  (2's comp), n_bits=8, bin_pt=6, quantization=Truncate, overflow=Wrap, period=1, timing_constraint=None, locs_specified=off, LOCs={}, needs_fixed_name=off, dbl_ovrd=off, show_param=off, xl_area=[0, 0, 0, 0, 0, 0, 0], xl_use_area=off}
      mask prompts: arith_type "Output Data Type"; n_bits "Number of Bits"; bin_pt "Binary Point"; period "Sample Period"; timing_constraint "IOB Timing Constraint"; locs_specified "Specify IOB Location Constraints"; LOCs "IOB Pad Locations (specify as cell array {'MSB', ..., 'LSB'})"; needs_fixed_name "Do Not Prepend Hierarchy to Port Name"; dbl_ovrd "Override with Double"; show_param "---------------------- Show Implementation Parameters -----------------------------------------------------------------------------------"; xl_area "FPGA Area [Slices, FFs, BRAMs, LUTs, IOBs, Emb. Mults, TBUFs]"; xl_use_area "Use Area Above For Estimation"
      mask help:
      | BLOCK IS OUT OF DATE.
      |
      | This block is from an outdated copy of the Xilinx Blockset. Please run xlUpdateModel('<model-name>') to update to the latest version.
      mask init:
      | [designRoot, family, part, speed, package, simulinkPeriod, sysclkPeriod, dbl_ovrd, trimVbit] = xlSysgenSettings(gcb,1,0);
      | trimVbit = 1;
      | [bg,fg] = xlcmap_r3('IO',dbl_ovrd);
      | iPos = get_param(gcb,'Position');
      | iWidth=iPos(3)-iPos(1); iHeight=iPos(4)-iPos(2);
      | iCx=iWidth/2;
      | iCy=iHeight/2;
      | [logoX, logoY] = xlogo(iPos);
      | 
      | 
      | nport = get_param(gcbh, 'ports');
      | nin = nport(1);
      | nout = nport(2);
      mask Help: eval('xlWeb(xlhtmldoclink(''Gateway In''))');
      mask StyleString: popup(Boolean|Unsigned|Signed  (2's comp)),edit,edit,popup(Truncate|Round  (unbiased: +/- Inf)),popup(Wrap|Saturate|Flag as Error),edit,popup(None|Data Rate|Data Rate;  Set 'FAST' Attribute),checkbox,edit,checkbox,checkbox,checkbox,edit,checkbox
      mask Display:
      | patch([0 iWidth iWidth 0],[0 0 iHeight iHeight] , bg);
      | patch(logoX,logoY , fg);
      | port_label('input',1,'dbl');
      | port_label('output',1,'fpt');
      | 
      | ;plot([0 0 iWidth iWidth 0], [0 iHeight iHeight 0 0]);
  Gateway Out : S-Function  FunctionName=xldeprecated  Parameters=nin,nout  mask(Xilinx Gateway Out){output_type=double, nbits=8, bin_pt=6, arith_type=Boolean, quantization=Truncate, overflow=Wrap, hdl_port=on, timing_constraint=None, locs_specified=off, LOCs={}, needs_fixed_name=off, show_param=off, xl_area=[0, 0, 0, 0, 0, 0, 0], xl_use_area=off}
      mask prompts: output_type "Output Data Type"; nbits "Number of Bits"; bin_pt "Binary Point"; arith_type "XFix Type"; hdl_port "Translate into Output Port"; timing_constraint "IOB Timing Constraint"; locs_specified "Specify IOB Location Constraints"; LOCs "IOB Pad Locations (cell array {'MSB', ..., 'LSB'})"; needs_fixed_name "Do Not Prepend Hierarchy to Port Name"; show_param "---------------------- Show Implementation Parameters -----------------------------------------------------------------------------------"; xl_area "FPGA Area [Slices, FFs, BRAMs, LUTs, IOBs, Emb. Mults, TBUFs]"; xl_use_area "Use Area Above For Estimation"
      mask help:
      | BLOCK IS OUT OF DATE.
      |
      | This block is from an outdated copy of the Xilinx Blockset. Please run xlUpdateModel('<model-name>') to update to the latest version.
      mask init:
      | [designRoot, family, part, speed, package, simulinkPeriod, sysclkPeriod, dbl_ovrd, trimVbit] = xlSysgenSettings(gcb,0,2);
      | [bg,fg] = xlcmap_r3('IO');
      | if (~hdl_port)
      |   [bg,fg]=xlcmap_r3('XBlock',1);
      | end
      | iPos = get_param(gcb,'Position');
      | iWidth=iPos(3)-iPos(1); iHeight=iPos(4)-iPos(2);
      | iCx=iWidth/2;
      | iCy=iHeight/2;
      | [logoX, logoY] = xlogo(iPos);
      | 
      | global xlfxdptinstalled
      | if isempty(xlfxdptinstalled)
      | 	v = ver('fixpoint');
      | 	xlfxdptinstalled = ~isempty(v);
      | end
      | nport = get_param(gcbh, 'ports');
      | nin = nport(1);
      | nout = nport(2);
      mask Help: eval('xlWeb(xlhtmldoclink(''Gateway Out''))');
      mask StyleString: popup(Automatic|Double|Integer|Simulink Fixed Point),edit,edit,popup(Boolean|Unsigned|Signed (2's comp)),popup(Truncate|Round (to +/-inf)),popup(Wrap|Saturate|Flag as Error),checkbox,popup(None|Data Rate|Data Rate;  Set 'FAST' Attribute),checkbox,edit,checkbox,checkbox,edit,checkbox
      mask Display:
      | patch([0 iWidth iWidth 0],[0 0 iHeight iHeight] , bg);
      | patch(logoX,logoY , fg);
      | port_label('input',1,'fpt');
      | port_label('output',1,'dbl');
      | 
      | ;plot([0 0 iWidth iWidth 0], [0 iHeight iHeight 0 0]);
  Indeterminate Probe : Subsystem  mask(Xilinx Indeterminate Probe){}
      mask help:
      | Indeterminate Probe.  Produces an output of type double that is 1 when input data is indeterminate.  Output is 0 otherwise.
      |
      | Hardware notes:  This block is ignored when hardware is generated.
      mask init:
      | [designRoot, family, part, speed, package, simulinkPeriod, sysclkPeriod, dbl_ovrd, trimVbit] = xlSysgenSettings(gcb,0,0);
      | 
      | [bg,fg] = xlcmap_r3('IO');
      | iPos = get_param(gcb,'Position');
      | iWidth=iPos(3)-iPos(1); iHeight=iPos(4)-iPos(2);
      | iCx=iWidth/2;
      | iCy=iHeight/2;
      | shapeX = iCx* (1 + cos(0:pi/6:2*pi));
      | shapeY = iCy* (1 + sin(0:pi/6:2*pi));
      settings: OpenFcn=modelName = get_param(bdroot, 'name');h = errordlg(sprintf(['This block is from an outdated copy of the Xilinx Blockset.\nPlease run xlUpdateModel(''' modelName ''') to update this design.']), 'Update Required');
      mask Help: eval('xlWeb(xlhtmldoclink(''Indeterminate Probe''))');
      mask Display:
      | patch(shapeX,shapeY, bg);
      | plot(shapeX,shapeY);
      | disp('!def');
  Interleaver Deinterleaver : S-Function  FunctionName=xldeprecated  Parameters=nin,nout  mask(Xilinx Interleaver/Deinterleaver){mode=Interleaver, num_branches=3, branch_length=[2 4 5], explicit_period=off, period=1, rst=off, en=off, dbl_ovrd=off, show_param=off, mem_type=Automatically Chosen, pipeline=off, use_rpm=on, gen_core=off, xl_area=[0, 0, 0, 0, 0, 0, 0], xl_use_area=off}
